simulink model "skarab_fgbe"  (R2016b)
settings: Solver=VariableStepDiscrete  StartTime=0.0  StopTime=50000  RelTol=1e-3
libraries: xbsIndex_r4 x558, casper_library_delays x131, xps_library x5, casper_library_misc x4
(part 3 of 7)

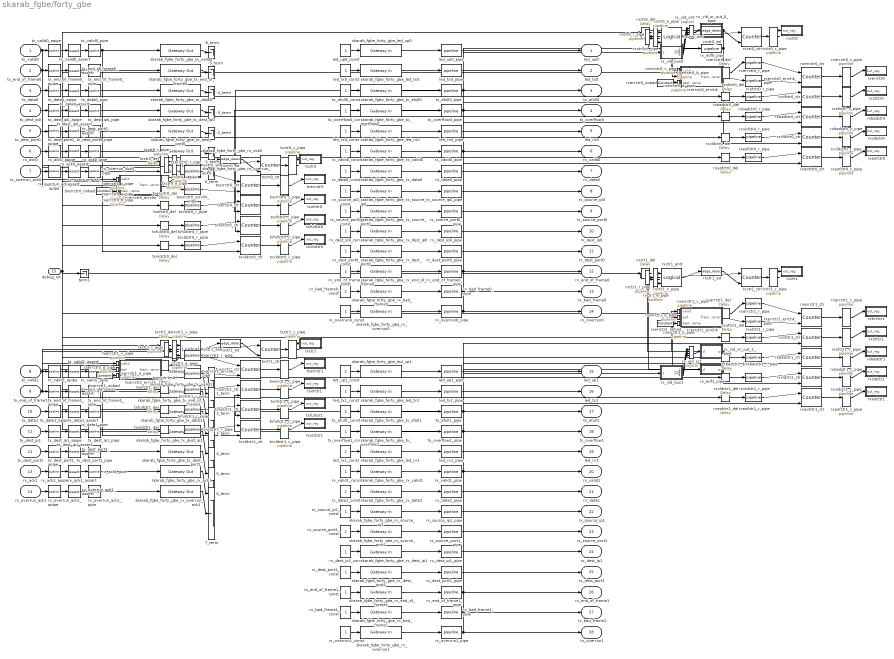
== system skarab_fgbe/forty_gbe ==
  tx_valid0 : Inport
  tx_end_of_frame0 : Inport  Port=2
  tx_data0 : Inport  Port=3
  tx_dest_ip0 : Inport  Port=4
  tx_dest_port0 : Inport  Port=5
  rx_ack0 : Inport  Port=6
  rx_overrun_ack0 : Inport  Port=7
  tx_valid1 : Inport  Port=8
  tx_end_of_frame1 : Inport  Port=9
  tx_data1 : Inport  Port=10
  tx_dest_ip1 : Inport  Port=11
  tx_dest_port1 : Inport  Port=12
  rx_ack1 : Inport  Port=13
  rx_overrun_ack1 : Inport  Port=14
  debug_rst : Inport  Port=15
  -1_term : Terminator
  -2_term : Terminator
  -3_term : Terminator
  -4_term : Terminator
  -5_term : Terminator
  -6_term : Terminator
  0_term : Terminator
  1_term : Terminator
  2_term : Terminator
  3_term : Terminator
  4_term : Terminator
  5_term : Terminator
  6_term : Terminator
  7_term : Terminator
  led_rx0_const : Constant
  led_rx0_pipe : casper_library_delays/pipeline  latency=3
      settings: AttributesFormatString=Latency = %<latency>
  led_rx1_const : Constant
  led_rx1_pipe : casper_library_delays/pipeline  latency=3
      settings: AttributesFormatString=Latency = %<latency>
  led_tx0_const : Constant
  led_tx0_pipe : casper_library_delays/pipeline  latency=3
      settings: AttributesFormatString=Latency = %<latency>
  led_tx1_const : Constant
  led_tx1_pipe : casper_library_delays/pipeline  latency=3
      settings: AttributesFormatString=Latency = %<latency>
  led_up0_const : Constant
  led_up0_pipe : casper_library_delays/pipeline  latency=3
      settings: AttributesFormatString=Latency = %<latency>
  led_up1_const : Constant
  led_up1_pipe : casper_library_delays/pipeline  latency=3
      settings: AttributesFormatString=Latency = %<latency>
  rx_ack0_apipe : casper_library_delays/pipeline  latency=3
      settings: AttributesFormatString=Latency = %<latency>
  rx_ack0_assert : xbsIndex_r4/Assert  assert_type=on  type_source=Explicitly  gui_display_data_type=Fixed-point  arith_type=Boolean  n_bits=1  bin_pt=0  preci_type=Single  exp_width=8  frac_width=24  assert_rate=on  rate_source=Explicitly  period=1  output_port=on  block_type=assert
  rx_ack0_pipe : casper_library_delays/pipeline  latency=3
      settings: AttributesFormatString=Latency = %<latency>
  rx_ack1_apipe : casper_library_delays/pipeline  latency=3
      settings: AttributesFormatString=Latency = %<latency>
  rx_ack1_assert : xbsIndex_r4/Assert  assert_type=on  type_source=Explicitly  gui_display_data_type=Fixed-point  arith_type=Boolean  n_bits=1  bin_pt=0  preci_type=Single  exp_width=8  frac_width=24  assert_rate=on  rate_source=Explicitly  period=1  output_port=on  block_type=assert
  rx_ack1_pipe : casper_library_delays/pipeline  latency=3
      settings: AttributesFormatString=Latency = %<latency>
  rx_bad_frame0_const : Constant
  rx_bad_frame0_pipe : casper_library_delays/pipeline  latency=3
      settings: AttributesFormatString=Latency = %<latency>
  rx_bad_frame1_const : Constant
  rx_bad_frame1_pipe : casper_library_delays/pipeline  latency=3
      settings: AttributesFormatString=Latency = %<latency>
  rx_data0_const : Constant
  rx_data0_pipe : casper_library_delays/pipeline  latency=3
      settings: AttributesFormatString=Latency = %<latency>
  rx_data1_const : Constant
  rx_data1_pipe : casper_library_delays/pipeline  latency=3
      settings: AttributesFormatString=Latency = %<latency>
  rx_dest_ip0_const : Constant
  rx_dest_ip0_pipe : casper_library_delays/pipeline  latency=3
      settings: AttributesFormatString=Latency = %<latency>
  rx_dest_ip1_const : Constant
  rx_dest_ip1_pipe : casper_library_delays/pipeline  latency=3
      settings: AttributesFormatString=Latency = %<latency>
  rx_dest_port0_const : Constant
  rx_dest_port0_pipe : casper_library_delays/pipeline  latency=3
      settings: AttributesFormatString=Latency = %<latency>
  rx_dest_port1_const : Constant
  rx_dest_port1_pipe : casper_library_delays/pipeline  latency=3
      settings: AttributesFormatString=Latency = %<latency>
  rx_end_of_frame0_const : Constant
  rx_end_of_frame0_pipe : casper_library_delays/pipeline  latency=3
      settings: AttributesFormatString=Latency = %<latency>
  rx_end_of_frame1_const : Constant
  rx_end_of_frame1_pipe : casper_library_delays/pipeline  latency=3
      settings: AttributesFormatString=Latency = %<latency>
  rx_eof0_pipe : casper_library_delays/pipeline  latency=3
      settings: AttributesFormatString=Latency = %<latency>
  rx_eof1_pipe : Subsystem  AncestorBlock=casper_library_delays/pipeline  mask(pipeline){latency=3}
      mask help:
      | An explicitly laid-out delay line to avoid mapping to SRL16s
      | for use in pipelining to help achieve timing closure.
      mask init:
      | pipeline_init(gcb,'latency',latency);
      settings: AttributesFormatString=Latency = %<latency>
      mask Display:
      | port_label('input', 1, 'd');
      | port_label('output', 1, 'q');
      | disp(['Z^-', num2str(latency)]);
  rx_overrun0_const : Constant
  rx_overrun0_pipe : casper_library_delays/pipeline  latency=3
      settings: AttributesFormatString=Latency = %<latency>
  rx_overrun1_const : Constant
  rx_overrun1_pipe : casper_library_delays/pipeline  latency=3
      settings: AttributesFormatString=Latency = %<latency>
  rx_overrun_ack0_apipe : casper_library_delays/pipeline  latency=3
      settings: AttributesFormatString=Latency = %<latency>
  rx_overrun_ack0_assert : xbsIndex_r4/Assert  assert_type=on  type_source=Explicitly  gui_display_data_type=Fixed-point  arith_type=Boolean  n_bits=1  bin_pt=0  preci_type=Single  exp_width=8  frac_width=24  assert_rate=on  rate_source=Explicitly  period=1  output_port=on  block_type=assert
  rx_overrun_ack0_pipe : casper_library_delays/pipeline  latency=3
      settings: AttributesFormatString=Latency = %<latency>
  rx_overrun_ack1_apipe : casper_library_delays/pipeline  latency=3
      settings: AttributesFormatString=Latency = %<latency>
  rx_overrun_ack1_assert : xbsIndex_r4/Assert  assert_type=on  type_source=Explicitly  gui_display_data_type=Fixed-point  arith_type=Boolean  n_bits=1  bin_pt=0  preci_type=Single  exp_width=8  frac_width=24  assert_rate=on  rate_source=Explicitly  period=1  output_port=on  block_type=assert
  rx_overrun_ack1_pipe : casper_library_delays/pipeline  latency=3
      settings: AttributesFormatString=Latency = %<latency>
  rx_source_ip0_const : Constant
  rx_source_ip0_pipe : casper_library_delays/pipeline  latency=3
      settings: AttributesFormatString=Latency = %<latency>
  rx_source_ip1_const : Constant
  rx_source_ip1_pipe : casper_library_delays/pipeline  latency=3
      settings: AttributesFormatString=Latency = %<latency>
  rx_source_port0_const : Constant
  rx_source_port0_pipe : casper_library_delays/pipeline  latency=3
      settings: AttributesFormatString=Latency = %<latency>
  rx_source_port1_const : Constant
  rx_source_port1_pipe : casper_library_delays/pipeline  latency=3
      settings: AttributesFormatString=Latency = %<latency>
  rx_valid0_const : Constant
  rx_valid0_pipe : casper_library_delays/pipeline  latency=3
      settings: AttributesFormatString=Latency = %<latency>
  rx_valid1_const : Constant
  rx_valid1_pipe : casper_library_delays/pipeline  latency=3
      settings: AttributesFormatString=Latency = %<latency>
  rx_vld_bus0 : Subsystem  AncestorBlock=casper_library_flow_control/bus_expand  mask(bus_expand){mode=divisions of equal size, outputNum=4, outputWidth=1, outputBinaryPt=0, outputArithmeticType=2, show_format=off, outputToWorkspace=off, variablePrefix=out, outputToModelAsWell=on}
      mask prompts: outputNum "Number of outputs:"; outputWidth "Output width:"; outputBinaryPt "Output binary point position:"; outputArithmeticType "Output arithmetic type (ufix=0, fix=1, bool=2):"; show_format "Print format string?"; outputToWorkspace "Output to workspace?"; variablePrefix "Variable name prefix:"; outputToModelAsWell "Output to model as well?"
      mask help:
      | Expands a 'bus' made using a bus_create or Xilinx
      | concat block.
      | The input will be divided into the specified number
      | of outputs with the specified arithmetic types.
      | Divisions are made from most significant bit.
      mask init:
      | bus_expand_init(gcb,...
      |     'mode', mode, ...
      |     'outputNum', outputNum, ...
      |     'outputWidth', outputWidth, ...
      |     'outputBinaryPt', outputBinaryPt, ...
      |     'outputArithmeticType', outputArithmeticType, ...
      |     'show_format', show_format, ...
      |     'outputToWorkspace', outputToWorkspace, ...
      |     'variablePrefix', variablePrefix, ...
      |     'outputToModelAsWell', outputToModelAsWell);
      settings: AttributesFormatString=4 outputs
      mask TypeOptions mode: divisions of equal size | divisions of arbitrary size
      mask Callback mode: bus_expand_callback();
      mask Callback outputWidth: bus_expand_callback();
      mask Callback outputToWorkspace: bus_expand_callback();
  rx_vld_bus1 : Subsystem  AncestorBlock=casper_library_flow_control/bus_expand  mask(bus_expand){mode=divisions of equal size, outputNum=4, outputWidth=1, outputBinaryPt=0, outputArithmeticType=2, show_format=off, outputToWorkspace=off, variablePrefix=out, outputToModelAsWell=on}
      mask prompts: outputNum "Number of outputs:"; outputWidth "Output width:"; outputBinaryPt "Output binary point position:"; outputArithmeticType "Output arithmetic type (ufix=0, fix=1, bool=2):"; show_format "Print format string?"; outputToWorkspace "Output to workspace?"; variablePrefix "Variable name prefix:"; outputToModelAsWell "Output to model as well?"
      mask help:
      | Expands a 'bus' made using a bus_create or Xilinx
      | concat block.
      | The input will be divided into the specified number
      | of outputs with the specified arithmetic types.
      | Divisions are made from most significant bit.
      mask init: same as skarab_fgbe/forty_gbe/rx_vld_bus0
      settings: AttributesFormatString=4 outputs
      mask TypeOptions mode: divisions of equal size | divisions of arbitrary size
      mask Callback mode: bus_expand_callback();
      mask Callback outputWidth: bus_expand_callback();
      mask Callback outputToWorkspace: bus_expand_callback();
  rx_vld_or0 : xbsIndex_r4/Logical  logical_function=OR  inputs=4  en=off  latency=1  precision=Full  arith_type=Unsigned  n_bits=16  bin_pt=0  align_bp=on  dbl_ovrd=off  block_type=logical
  rx_vld_or1 : xbsIndex_r4/Logical  logical_function=OR  inputs=4  en=off  latency=1  precision=Full  arith_type=Unsigned  n_bits=16  bin_pt=0  align_bp=on  dbl_ovrd=off  block_type=logical
  rx_vld_or_out_0_pipe : Subsystem  AncestorBlock=casper_library_delays/pipeline  mask(pipeline){latency=2}
      mask help:
      | An explicitly laid-out delay line to avoid mapping to SRL16s
      | for use in pipelining to help achieve timing closure.
      mask init:
      | pipeline_init(gcb,'latency',latency);
      settings: AttributesFormatString=Latency = %<latency>
      mask Display:
      | port_label('input', 1, 'd');
      | port_label('output', 1, 'q');
      | disp(['Z^-', num2str(latency)]);
  rx_vld_or_out_1_pipe : Subsystem  AncestorBlock=casper_library_delays/pipeline  mask(pipeline){latency=2}
      mask help:
      | An explicitly laid-out delay line to avoid mapping to SRL16s
      | for use in pipelining to help achieve timing closure.
      mask init:
      | pipeline_init(gcb,'latency',latency);
      settings: AttributesFormatString=Latency = %<latency>
      mask Display:
      | port_label('input', 1, 'd');
      | port_label('output', 1, 'q');
      | disp(['Z^-', num2str(latency)]);
  rxbadctr0 : Subsystem  Tag=xps:sw_reg  AncestorBlock=xps_library/Memory/software_register  mask(swreg){io_dir=To Processor, io_delay=1, init_val=0, sample_period=1, names=reg, bitwidths=16, bin_pts=0, arith_types=0, sim_port=off, show_format=on}
      mask prompts: io_dir "I/O direction"; io_delay "I/O delay"; init_val "Initial Value"; sample_period "Sample period"; names "Bitfield names [msb...lsb]"; bitwidths "Bitfield widths"; bin_pts "Bitfield binary pts"; arith_types "Bitfield types, ufix=0, fix=1, bool=2"; sim_port "Provide sim input/output?"; show_format "Print format string?"
      mask help: A 32-bit software-accessible register. Can be divided into bitfields of varying widths and types using the fields in the block mask.
      mask init:
      | swreg_init(gcb)
      settings: AttributesFormatString=1output:uf16.0 = 16 bits
      mask TypeOptions io_dir: To Processor | From Processor
      mask Callback io_dir:
      | mask_enables = get_param(gcb, 'MaskEnables');
      | mask_names = get_param(gcb, 'MaskNames');
      | if strcmp(get_param(gcb, 'io_dir'), 'To Processor'),
      |     mask_enables{ismember(mask_names, 'sample_period')} = 'off';
      | else
      |     mask_enables{ismember(mask_names, 'sample_period')} = 'on';
      | end
      | set_param(gcb, 'MaskEnables', mask_enables);
      mask DialogControl ParameterTabVar0 Prompt: Setup
  rxbadctr0_c_pipe : casper_library_delays/pipeline  latency=3
      settings: AttributesFormatString=Latency = %<latency>
  rxbadctr0_ctr : xbsIndex_r4/Counter  cnt_type=Free Running  cnt_to=Inf  operation=Up  start_count=0  cnt_by_val=1  arith_type=Unsigned  n_bits=16  bin_pt=0  load_pin=off  rst=on  en=on  explicit_period=on  period=1  use_behavioral_HDL=on  implementation=Fabric  dbl_ovrd=off  block_type=counter
  rxbadctr0_del : xbsIndex_r4/Delay  rst=off  infoeditControl=Selection of Reset will increase slice count due to use of real FFs and instead of SRLs  en=off  latency=1  reg_retiming=on  dbl_ovrd=off  block_type=delay
      settings: infoedit=Hardware notes: A delay line is a chain, each link of which is an SRL16 or SRL32 followed by a flip-flop.
  rxbadctr0_r_pipe : casper_library_delays/pipeline  latency=3
      settings: AttributesFormatString=Latency = %<latency>
  rxbadctr1 : Subsystem  Tag=xps:sw_reg  AncestorBlock=xps_library/Memory/software_register  mask(swreg){io_dir=To Processor, io_delay=1, init_val=0, sample_period=1, names=reg, bitwidths=16, bin_pts=0, arith_types=0, sim_port=off, show_format=on}
      mask prompts: io_dir "I/O direction"; io_delay "I/O delay"; init_val "Initial Value"; sample_period "Sample period"; names "Bitfield names [msb...lsb]"; bitwidths "Bitfield widths"; bin_pts "Bitfield binary pts"; arith_types "Bitfield types, ufix=0, fix=1, bool=2"; sim_port "Provide sim input/output?"; show_format "Print format string?"
      mask help: A 32-bit software-accessible register. Can be divided into bitfields of varying widths and types using the fields in the block mask.
      mask init:
      | swreg_init(gcb)
      settings: AttributesFormatString=1output:uf16.0 = 16 bits
      mask TypeOptions io_dir: To Processor | From Processor
      mask Callback io_dir:
      | mask_enables = get_param(gcb, 'MaskEnables');
      | mask_names = get_param(gcb, 'MaskNames');
      | if strcmp(get_param(gcb, 'io_dir'), 'To Processor'),
      |     mask_enables{ismember(mask_names, 'sample_period')} = 'off';
      | else
      |     mask_enables{ismember(mask_names, 'sample_period')} = 'on';
      | end
      | set_param(gcb, 'MaskEnables', mask_enables);
      mask DialogControl ParameterTabVar0 Prompt: Setup
  rxbadctr1_c_pipe : casper_library_delays/pipeline  latency=3
      settings: AttributesFormatString=Latency = %<latency>
  rxbadctr1_ctr : xbsIndex_r4/Counter  cnt_type=Free Running  cnt_to=Inf  operation=Up  start_count=0  cnt_by_val=1  arith_type=Unsigned  n_bits=16  bin_pt=0  load_pin=off  rst=on  en=on  explicit_period=on  period=1  use_behavioral_HDL=on  implementation=Fabric  dbl_ovrd=off  block_type=counter
  rxbadctr1_del : xbsIndex_r4/Delay  rst=off  infoeditControl=Selection of Reset will increase slice count due to use of real FFs and instead of SRLs  en=off  latency=1  reg_retiming=on  dbl_ovrd=off  block_type=delay
      settings: infoedit=Hardware notes: A delay line is a chain, each link of which is an SRL16 or SRL32 followed by a flip-flop.
  rxbadctr1_r_pipe : casper_library_delays/pipeline  latency=3
      settings: AttributesFormatString=Latency = %<latency>
  rxctr0 : Subsystem  Tag=xps:sw_reg  AncestorBlock=xps_library/Memory/software_register  mask(swreg){io_dir=To Processor, io_delay=1, init_val=0, sample_period=1, names=reg, bitwidths=16, bin_pts=0, arith_types=0, sim_port=off, show_format=on}
      mask prompts: io_dir "I/O direction"; io_delay "I/O delay"; init_val "Initial Value"; sample_period "Sample period"; names "Bitfield names [msb...lsb]"; bitwidths "Bitfield widths"; bin_pts "Bitfield binary pts"; arith_types "Bitfield types, ufix=0, fix=1, bool=2"; sim_port "Provide sim input/output?"; show_format "Print format string?"
      mask help: A 32-bit software-accessible register. Can be divided into bitfields of varying widths and types using the fields in the block mask.
      mask init:
      | swreg_init(gcb)
      settings: AttributesFormatString=1output:uf16.0 = 16 bits
      mask TypeOptions io_dir: To Processor | From Processor
      mask Callback io_dir:
      | mask_enables = get_param(gcb, 'MaskEnables');
      | mask_names = get_param(gcb, 'MaskNames');
      | if strcmp(get_param(gcb, 'io_dir'), 'To Processor'),
      |     mask_enables{ismember(mask_names, 'sample_period')} = 'off';
      | else
      |     mask_enables{ismember(mask_names, 'sample_period')} = 'on';
      | end
      | set_param(gcb, 'MaskEnables', mask_enables);
      mask DialogControl ParameterTabVar0 Prompt: Setup
  rxctr0_and : xbsIndex_r4/Logical  logical_function=AND  inputs=2  en=off  latency=1  precision=Full  arith_type=Unsigned  n_bits=16  bin_pt=0  align_bp=on  dbl_ovrd=off  block_type=logical
  rxctr0_c_pipe : casper_library_delays/pipeline  latency=3
      settings: AttributesFormatString=Latency = %<latency>
  rxctr0_ctr : xbsIndex_r4/Counter  cnt_type=Free Running  cnt_to=Inf  operation=Up  start_count=0  cnt_by_val=1  arith_type=Unsigned  n_bits=16  bin_pt=0  load_pin=off  rst=on  en=on  explicit_period=on  period=1  use_behavioral_HDL=on  implementation=Fabric  dbl_ovrd=off  block_type=counter
  rxctr0_del : xbsIndex_r4/Delay  rst=off  infoeditControl=Selection of Reset will increase slice count due to use of real FFs and instead of SRLs  en=off  latency=1  reg_retiming=on  dbl_ovrd=off  block_type=delay
      settings: infoedit=Hardware notes: A delay line is a chain, each link of which is an SRL16 or SRL32 followed by a flip-flop.
  rxctr0_e_pipe : casper_library_delays/pipeline  latency=3
      settings: AttributesFormatString=Latency = %<latency>
  rxctr0_ed : casper_library_misc/edge_detect  edge=Rising  polarity=Active High  x_in=[0 0.08 0.08 0.16 0.16 0.24 0.24 0.32 0.32 0.4]  y_in="[-1 -1  1  1  1  1  1  1  1  1]"  x_out=[0.6 0.68 0.68 0.76 0.76 0.84 0.84 0.92 0.92 1]  y_out="[-1 -1  1  1 -1 -1 -1 -1 -1 -1]"
  rxctr0_r_pipe : casper_library_delays/pipeline  latency=3
      settings: AttributesFormatString=Latency = %<latency>
  rxctr0_v_pipe : casper_library_delays/pipeline  latency=3
      settings: AttributesFormatString=Latency = %<latency>
  rxctr1 : Subsystem  Tag=xps:sw_reg  AncestorBlock=xps_library/Memory/software_register  mask(swreg){io_dir=To Processor, io_delay=1, init_val=0, sample_period=1, names=reg, bitwidths=16, bin_pts=0, arith_types=0, sim_port=off, show_format=on}
      mask prompts: io_dir "I/O direction"; io_delay "I/O delay"; init_val "Initial Value"; sample_period "Sample period"; names "Bitfield names [msb...lsb]"; bitwidths "Bitfield widths"; bin_pts "Bitfield binary pts"; arith_types "Bitfield types, ufix=0, fix=1, bool=2"; sim_port "Provide sim input/output?"; show_format "Print format string?"
      mask help: A 32-bit software-accessible register. Can be divided into bitfields of varying widths and types using the fields in the block mask.
      mask init:
      | swreg_init(gcb)
      settings: AttributesFormatString=1output:uf16.0 = 16 bits
      mask TypeOptions io_dir: To Processor | From Processor
      mask Callback io_dir:
      | mask_enables = get_param(gcb, 'MaskEnables');
      | mask_names = get_param(gcb, 'MaskNames');
      | if strcmp(get_param(gcb, 'io_dir'), 'To Processor'),
      |     mask_enables{ismember(mask_names, 'sample_period')} = 'off';
      | else
      |     mask_enables{ismember(mask_names, 'sample_period')} = 'on';
      | end
      | set_param(gcb, 'MaskEnables', mask_enables);
      mask DialogControl ParameterTabVar0 Prompt: Setup
  rxctr1_and : xbsIndex_r4/Logical  logical_function=AND  inputs=2  en=off  latency=1  precision=Full  arith_type=Unsigned  n_bits=16  bin_pt=0  align_bp=on  dbl_ovrd=off  block_type=logical
  rxctr1_c_pipe : casper_library_delays/pipeline  latency=3
      settings: AttributesFormatString=Latency = %<latency>
  rxctr1_ctr : xbsIndex_r4/Counter  cnt_type=Free Running  cnt_to=Inf  operation=Up  start_count=0  cnt_by_val=1  arith_type=Unsigned  n_bits=16  bin_pt=0  load_pin=off  rst=on  en=on  explicit_period=on  period=1  use_behavioral_HDL=on  implementation=Fabric  dbl_ovrd=off  block_type=counter
  rxctr1_del : xbsIndex_r4/Delay  rst=off  infoeditControl=Selection of Reset will increase slice count due to use of real FFs and instead of SRLs  en=off  latency=1  reg_retiming=on  dbl_ovrd=off  block_type=delay
      settings: infoedit=Hardware notes: A delay line is a chain, each link of which is an SRL16 or SRL32 followed by a flip-flop.
  rxctr1_e_pipe : casper_library_delays/pipeline  latency=3
      settings: AttributesFormatString=Latency = %<latency>
  rxctr1_ed : casper_library_misc/edge_detect  edge=Rising  polarity=Active High  x_in=[0 0.08 0.08 0.16 0.16 0.24 0.24 0.32 0.32 0.4]  y_in="[-1 -1  1  1  1  1  1  1  1  1]"  x_out=[0.6 0.68 0.68 0.76 0.76 0.84 0.84 0.92 0.92 1]  y_out="[-1 -1  1  1 -1 -1 -1 -1 -1 -1]"
  rxctr1_r_pipe : casper_library_delays/pipeline  latency=3
      settings: AttributesFormatString=Latency = %<latency>
  rxctr1_v_pipe : casper_library_delays/pipeline  latency=3
      settings: AttributesFormatString=Latency = %<latency>
  rxeofctr0 : Subsystem  Tag=xps:sw_reg  AncestorBlock=xps_library/Memory/software_register  mask(swreg){io_dir=To Processor, io_delay=1, init_val=0, sample_period=1, names=reg, bitwidths=16, bin_pts=0, arith_types=0, sim_port=off, show_format=on}
      mask prompts: io_dir "I/O direction"; io_delay "I/O delay"; init_val "Initial Value"; sample_period "Sample period"; names "Bitfield names [msb...lsb]"; bitwidths "Bitfield widths"; bin_pts "Bitfield binary pts"; arith_types "Bitfield types, ufix=0, fix=1, bool=2"; sim_port "Provide sim input/output?"; show_format "Print format string?"
      mask help: A 32-bit software-accessible register. Can be divided into bitfields of varying widths and types using the fields in the block mask.
      mask init:
      | swreg_init(gcb)
      settings: AttributesFormatString=1output:uf16.0 = 16 bits
      mask TypeOptions io_dir: To Processor | From Processor
      mask Callback io_dir:
      | mask_enables = get_param(gcb, 'MaskEnables');
      | mask_names = get_param(gcb, 'MaskNames');
      | if strcmp(get_param(gcb, 'io_dir'), 'To Processor'),
      |     mask_enables{ismember(mask_names, 'sample_period')} = 'off';
      | else
      |     mask_enables{ismember(mask_names, 'sample_period')} = 'on';
      | end
      | set_param(gcb, 'MaskEnables', mask_enables);
      mask DialogControl ParameterTabVar0 Prompt: Setup
  rxeofctr0_c_pipe : casper_library_delays/pipeline  latency=3
      settings: AttributesFormatString=Latency = %<latency>
  rxeofctr0_ctr : xbsIndex_r4/Counter  cnt_type=Free Running  cnt_to=Inf  operation=Up  start_count=0  cnt_by_val=1  arith_type=Unsigned  n_bits=16  bin_pt=0  load_pin=off  rst=on  en=on  explicit_period=on  period=1  use_behavioral_HDL=on  implementation=Fabric  dbl_ovrd=off  block_type=counter
  rxeofctr0_del : xbsIndex_r4/Delay  rst=off  infoeditControl=Selection of Reset will increase slice count due to use of real FFs and instead of SRLs  en=off  latency=1  reg_retiming=on  dbl_ovrd=off  block_type=delay
      settings: infoedit=Hardware notes: A delay line is a chain, each link of which is an SRL16 or SRL32 followed by a flip-flop.
  rxeofctr0_r_pipe : casper_library_delays/pipeline  latency=3
      settings: AttributesFormatString=Latency = %<latency>
  rxeofctr1 : Subsystem  Tag=xps:sw_reg  AncestorBlock=xps_library/Memory/software_register  mask(swreg){io_dir=To Processor, io_delay=1, init_val=0, sample_period=1, names=reg, bitwidths=16, bin_pts=0, arith_types=0, sim_port=off, show_format=on}
      mask prompts: io_dir "I/O direction"; io_delay "I/O delay"; init_val "Initial Value"; sample_period "Sample period"; names "Bitfield names [msb...lsb]"; bitwidths "Bitfield widths"; bin_pts "Bitfield binary pts"; arith_types "Bitfield types, ufix=0, fix=1, bool=2"; sim_port "Provide sim input/output?"; show_format "Print format string?"
      mask help: A 32-bit software-accessible register. Can be divided into bitfields of varying widths and types using the fields in the block mask.
      mask init:
      | swreg_init(gcb)
      settings: AttributesFormatString=1output:uf16.0 = 16 bits
      mask TypeOptions io_dir: To Processor | From Processor
      mask Callback io_dir:
      | mask_enables = get_param(gcb, 'MaskEnables');
      | mask_names = get_param(gcb, 'MaskNames');
      | if strcmp(get_param(gcb, 'io_dir'), 'To Processor'),
      |     mask_enables{ismember(mask_names, 'sample_period')} = 'off';
      | else
      |     mask_enables{ismember(mask_names, 'sample_period')} = 'on';
      | end
      | set_param(gcb, 'MaskEnables', mask_enables);
      mask DialogControl ParameterTabVar0 Prompt: Setup
  rxeofctr1_c_pipe : casper_library_delays/pipeline  latency=3
      settings: AttributesFormatString=Latency = %<latency>
  rxeofctr1_ctr : xbsIndex_r4/Counter  cnt_type=Free Running  cnt_to=Inf  operation=Up  start_count=0  cnt_by_val=1  arith_type=Unsigned  n_bits=16  bin_pt=0  load_pin=off  rst=on  en=on  explicit_period=on  period=1  use_behavioral_HDL=on  implementation=Fabric  dbl_ovrd=off  block_type=counter
  rxeofctr1_del : xbsIndex_r4/Delay  rst=off  infoeditControl=Selection of Reset will increase slice count due to use of real FFs and instead of SRLs  en=off  latency=1  reg_retiming=on  dbl_ovrd=off  block_type=delay
      settings: infoedit=Hardware notes: A delay line is a chain, each link of which is an SRL16 or SRL32 followed by a flip-flop.
  rxeofctr1_r_pipe : casper_library_delays/pipeline  latency=3
      settings: AttributesFormatString=Latency = %<latency>
  rxerrctr0 : Subsystem  Tag=xps:sw_reg  AncestorBlock=xps_library/Memory/software_register  mask(swreg){io_dir=To Processor, io_delay=1, init_val=0, sample_period=1, names=reg, bitwidths=16, bin_pts=0, arith_types=0, sim_port=off, show_format=on}
      mask prompts: io_dir "I/O direction"; io_delay "I/O delay"; init_val "Initial Value"; sample_period "Sample period"; names "Bitfield names [msb...lsb]"; bitwidths "Bitfield widths"; bin_pts "Bitfield binary pts"; arith_types "Bitfield types, ufix=0, fix=1, bool=2"; sim_port "Provide sim input/output?"; show_format "Print format string?"
      mask help: A 32-bit software-accessible register. Can be divided into bitfields of varying widths and types using the fields in the block mask.
      mask init:
      | swreg_init(gcb)
      settings: AttributesFormatString=1output:uf16.0 = 16 bits
      mask TypeOptions io_dir: To Processor | From Processor
      mask Callback io_dir:
      | mask_enables = get_param(gcb, 'MaskEnables');
      | mask_names = get_param(gcb, 'MaskNames');
      | if strcmp(get_param(gcb, 'io_dir'), 'To Processor'),
      |     mask_enables{ismember(mask_names, 'sample_period')} = 'off';
      | else
      |     mask_enables{ismember(mask_names, 'sample_period')} = 'on';
      | end
      | set_param(gcb, 'MaskEnables', mask_enables);
      mask DialogControl ParameterTabVar0 Prompt: Setup
  rxerrctr0_b_pipe : casper_library_delays/pipeline  latency=3
      settings: AttributesFormatString=Latency = %<latency>
  rxerrctr0_c_pipe : casper_library_delays/pipeline  latency=3
      settings: AttributesFormatString=Latency = %<latency>
  rxerrctr0_ctr : xbsIndex_r4/Counter  cnt_type=Free Running  cnt_to=Inf  operation=Up  start_count=0  cnt_by_val=1  arith_type=Unsigned  n_bits=16  bin_pt=0  load_pin=off  rst=on  en=on  explicit_period=on  period=1  use_behavioral_HDL=on  implementation=Fabric  dbl_ovrd=off  block_type=counter
  rxerrctr0_del : xbsIndex_r4/Delay  rst=off  infoeditControl=Selection of Reset will increase slice count due to use of real FFs and instead of SRLs  en=off  latency=1  reg_retiming=on  dbl_ovrd=off  block_type=delay
      settings: infoedit=Hardware notes: A delay line is a chain, each link of which is an SRL16 or SRL32 followed by a flip-flop.
  rxerrctr0_e_pipe : casper_library_delays/pipeline  latency=3
      settings: AttributesFormatString=Latency = %<latency>
  rxerrctr0_errchk : Subsystem  Tag=casper:frame_len_checker  AncestorBlock=casper_library_communications/frame_len_checker  mask{frame_len=100}
      mask prompts: frame_len "Frame length (64-bit words):"
      mask help: Monitors valid, EOF and bad_frame signals in/from a 10Gbe core and outputs an error signal. Can be used to drive an error counter or latched as a flag.
  rxerrctr0_errchk_pipe : casper_library_delays/pipeline  latency=3
      settings: AttributesFormatString=Latency = %<latency>
  rxerrctr0_nobad : xbsIndex_r4/Constant  const=0  gui_display_data_type=Fixed-point  arith_type=Boolean  n_bits=16  bin_pt=14  preci_type=Single  exp_width=8  frac_width=24  explicit_period=on  period=1  equ=P=C  opselect=C  inp2=PCIN>>17  opr=+  inp1=P  carry=CIN  dbl_ovrd=off  block_type=constant
  rxerrctr0_r_pipe : casper_library_delays/pipeline  latency=3
      settings: AttributesFormatString=Latency = %<latency>
  rxerrctr0_v_pipe : casper_library_delays/pipeline  latency=3
      settings: AttributesFormatString=Latency = %<latency>
  rxerrctr1 : Subsystem  Tag=xps:sw_reg  AncestorBlock=xps_library/Memory/software_register  mask(swreg){io_dir=To Processor, io_delay=1, init_val=0, sample_period=1, names=reg, bitwidths=16, bin_pts=0, arith_types=0, sim_port=off, show_format=on}
      mask prompts: io_dir "I/O direction"; io_delay "I/O delay"; init_val "Initial Value"; sample_period "Sample period"; names "Bitfield names [msb...lsb]"; bitwidths "Bitfield widths"; bin_pts "Bitfield binary pts"; arith_types "Bitfield types, ufix=0, fix=1, bool=2"; sim_port "Provide sim input/output?"; show_format "Print format string?"
      mask help: A 32-bit software-accessible register. Can be divided into bitfields of varying widths and types using the fields in the block mask.
      mask init:
      | swreg_init(gcb)
      settings: AttributesFormatString=1output:uf16.0 = 16 bits
      mask TypeOptions io_dir: To Processor | From Processor
      mask Callback io_dir:
      | mask_enables = get_param(gcb, 'MaskEnables');
      | mask_names = get_param(gcb, 'MaskNames');
      | if strcmp(get_param(gcb, 'io_dir'), 'To Processor'),
      |     mask_enables{ismember(mask_names, 'sample_period')} = 'off';
      | else
      |     mask_enables{ismember(mask_names, 'sample_period')} = 'on';
      | end
      | set_param(gcb, 'MaskEnables', mask_enables);
      mask DialogControl ParameterTabVar0 Prompt: Setup
  rxerrctr1_b_pipe : casper_library_delays/pipeline  latency=3
      settings: AttributesFormatString=Latency = %<latency>
  rxerrctr1_c_pipe : casper_library_delays/pipeline  latency=3
      settings: AttributesFormatString=Latency = %<latency>
  rxerrctr1_ctr : xbsIndex_r4/Counter  cnt_type=Free Running  cnt_to=Inf  operation=Up  start_count=0  cnt_by_val=1  arith_type=Unsigned  n_bits=16  bin_pt=0  load_pin=off  rst=on  en=on  explicit_period=on  period=1  use_behavioral_HDL=on  implementation=Fabric  dbl_ovrd=off  block_type=counter
  rxerrctr1_del : xbsIndex_r4/Delay  rst=off  infoeditControl=Selection of Reset will increase slice count due to use of real FFs and instead of SRLs  en=off  latency=1  reg_retiming=on  dbl_ovrd=off  block_type=delay
      settings: infoedit=Hardware notes: A delay line is a chain, each link of which is an SRL16 or SRL32 followed by a flip-flop.
  rxerrctr1_e_pipe : casper_library_delays/pipeline  latency=3
      settings: AttributesFormatString=Latency = %<latency>
  rxerrctr1_errchk : Subsystem  Tag=casper:frame_len_checker  AncestorBlock=casper_library_communications/frame_len_checker  mask{frame_len=100}
      mask prompts: frame_len "Frame length (64-bit words):"
      mask help: Monitors valid, EOF and bad_frame signals in/from a 10Gbe core and outputs an error signal. Can be used to drive an error counter or latched as a flag.
  rxerrctr1_errchk_pipe : casper_library_delays/pipeline  latency=3
      settings: AttributesFormatString=Latency = %<latency>
  rxerrctr1_nobad : xbsIndex_r4/Constant  const=0  gui_display_data_type=Fixed-point  arith_type=Boolean  n_bits=16  bin_pt=14  preci_type=Single  exp_width=8  frac_width=24  explicit_period=on  period=1  equ=P=C  opselect=C  inp2=PCIN>>17  opr=+  inp1=P  carry=CIN  dbl_ovrd=off  block_type=constant
  rxerrctr1_r_pipe : casper_library_delays/pipeline  latency=3
      settings: AttributesFormatString=Latency = %<latency>
  rxerrctr1_v_pipe : casper_library_delays/pipeline  latency=3
      settings: AttributesFormatString=Latency = %<latency>
  rxofctr0 : Subsystem  Tag=xps:sw_reg  AncestorBlock=xps_library/Memory/software_register  mask(swreg){io_dir=To Processor, io_delay=1, init_val=0, sample_period=1, names=reg, bitwidths=16, bin_pts=0, arith_types=0, sim_port=off, show_format=on}
      mask prompts: io_dir "I/O direction"; io_delay "I/O delay"; init_val "Initial Value"; sample_period "Sample period"; names "Bitfield names [msb...lsb]"; bitwidths "Bitfield widths"; bin_pts "Bitfield binary pts"; arith_types "Bitfield types, ufix=0, fix=1, bool=2"; sim_port "Provide sim input/output?"; show_format "Print format string?"
      mask help: A 32-bit software-accessible register. Can be divided into bitfields of varying widths and types using the fields in the block mask.
      mask init:
      | swreg_init(gcb)
      settings: AttributesFormatString=1output:uf16.0 = 16 bits
      mask TypeOptions io_dir: To Processor | From Processor
      mask Callback io_dir:
      | mask_enables = get_param(gcb, 'MaskEnables');
      | mask_names = get_param(gcb, 'MaskNames');
      | if strcmp(get_param(gcb, 'io_dir'), 'To Processor'),
      |     mask_enables{ismember(mask_names, 'sample_period')} = 'off';
      | else
      |     mask_enables{ismember(mask_names, 'sample_period')} = 'on';
      | end
      | set_param(gcb, 'MaskEnables', mask_enables);
      mask DialogControl ParameterTabVar0 Prompt: Setup
  rxofctr0_c_pipe : casper_library_delays/pipeline  latency=3
      settings: AttributesFormatString=Latency = %<latency>
  rxofctr0_ctr : xbsIndex_r4/Counter  cnt_type=Free Running  cnt_to=Inf  operation=Up  start_count=0  cnt_by_val=1  arith_type=Unsigned  n_bits=16  bin_pt=0  load_pin=off  rst=on  en=on  explicit_period=on  period=1  use_behavioral_HDL=on  implementation=Fabric  dbl_ovrd=off  block_type=counter
  rxofctr0_del : xbsIndex_r4/Delay  rst=off  infoeditControl=Selection of Reset will increase slice count due to use of real FFs and instead of SRLs  en=off  latency=1  reg_retiming=on  dbl_ovrd=off  block_type=delay
      settings: infoedit=Hardware notes: A delay line is a chain, each link of which is an SRL16 or SRL32 followed by a flip-flop.
  rxofctr0_r_pipe : casper_library_delays/pipeline  latency=3
      settings: AttributesFormatString=Latency = %<latency>
  rxofctr1 : Subsystem  Tag=xps:sw_reg  AncestorBlock=xps_library/Memory/software_register  mask(swreg){io_dir=To Processor, io_delay=1, init_val=0, sample_period=1, names=reg, bitwidths=16, bin_pts=0, arith_types=0, sim_port=off, show_format=on}
      mask prompts: io_dir "I/O direction"; io_delay "I/O delay"; init_val "Initial Value"; sample_period "Sample period"; names "Bitfield names [msb...lsb]"; bitwidths "Bitfield widths"; bin_pts "Bitfield binary pts"; arith_types "Bitfield types, ufix=0, fix=1, bool=2"; sim_port "Provide sim input/output?"; show_format "Print format string?"
      mask help: A 32-bit software-accessible register. Can be divided into bitfields of varying widths and types using the fields in the block mask.
      mask init:
      | swreg_init(gcb)
      settings: AttributesFormatString=1output:uf16.0 = 16 bits
      mask TypeOptions io_dir: To Processor | From Processor
      mask Callback io_dir:
      | mask_enables = get_param(gcb, 'MaskEnables');
      | mask_names = get_param(gcb, 'MaskNames');
      | if strcmp(get_param(gcb, 'io_dir'), 'To Processor'),
      |     mask_enables{ismember(mask_names, 'sample_period')} = 'off';
      | else
      |     mask_enables{ismember(mask_names, 'sample_period')} = 'on';
      | end
      | set_param(gcb, 'MaskEnables', mask_enables);
      mask DialogControl ParameterTabVar0 Prompt: Setup
  rxofctr1_c_pipe : casper_library_delays/pipeline  latency=3
      settings: AttributesFormatString=Latency = %<latency>
  rxofctr1_ctr : xbsIndex_r4/Counter  cnt_type=Free Running  cnt_to=Inf  operation=Up  start_count=0  cnt_by_val=1  arith_type=Unsigned  n_bits=16  bin_pt=0  load_pin=off  rst=on  en=on  explicit_period=on  period=1  use_behavioral_HDL=on  implementation=Fabric  dbl_ovrd=off  block_type=counter
  rxofctr1_del : xbsIndex_r4/Delay  rst=off  infoeditControl=Selection of Reset will increase slice count due to use of real FFs and instead of SRLs  en=off  latency=1  reg_retiming=on  dbl_ovrd=off  block_type=delay
      settings: infoedit=Hardware notes: A delay line is a chain, each link of which is an SRL16 or SRL32 followed by a flip-flop.
  rxofctr1_r_pipe : casper_library_delays/pipeline  latency=3
      settings: AttributesFormatString=Latency = %<latency>
  rxvldctr0 : Subsystem  Tag=xps:sw_reg  AncestorBlock=xps_library/Memory/software_register  mask(swreg){io_dir=To Processor, io_delay=1, init_val=0, sample_period=1, names=reg, bitwidths=16, bin_pts=0, arith_types=0, sim_port=off, show_format=on}
      mask prompts: io_dir "I/O direction"; io_delay "I/O delay"; init_val "Initial Value"; sample_period "Sample period"; names "Bitfield names [msb...lsb]"; bitwidths "Bitfield widths"; bin_pts "Bitfield binary pts"; arith_types "Bitfield types, ufix=0, fix=1, bool=2"; sim_port "Provide sim input/output?"; show_format "Print format string?"
      mask help: A 32-bit software-accessible register. Can be divided into bitfields of varying widths and types using the fields in the block mask.
      mask init:
      | swreg_init(gcb)
      settings: AttributesFormatString=1output:uf16.0 = 16 bits
      mask TypeOptions io_dir: To Processor | From Processor
      mask Callback io_dir:
      | mask_enables = get_param(gcb, 'MaskEnables');
      | mask_names = get_param(gcb, 'MaskNames');
      | if strcmp(get_param(gcb, 'io_dir'), 'To Processor'),
      |     mask_enables{ismember(mask_names, 'sample_period')} = 'off';
      | else
      |     mask_enables{ismember(mask_names, 'sample_period')} = 'on';
      | end
      | set_param(gcb, 'MaskEnables', mask_enables);
      mask DialogControl ParameterTabVar0 Prompt: Setup
  rxvldctr0_c_pipe : casper_library_delays/pipeline  latency=3
      settings: AttributesFormatString=Latency = %<latency>
  rxvldctr0_ctr : xbsIndex_r4/Counter  cnt_type=Free Running  cnt_to=Inf  operation=Up  start_count=0  cnt_by_val=1  arith_type=Unsigned  n_bits=16  bin_pt=0  load_pin=off  rst=on  en=on  explicit_period=on  period=1  use_behavioral_HDL=on  implementation=Fabric  dbl_ovrd=off  block_type=counter
  rxvldctr0_del : xbsIndex_r4/Delay  rst=off  infoeditControl=Selection of Reset will increase slice count due to use of real FFs and instead of SRLs  en=off  latency=1  reg_retiming=on  dbl_ovrd=off  block_type=delay
      settings: infoedit=Hardware notes: A delay line is a chain, each link of which is an SRL16 or SRL32 followed by a flip-flop.
  rxvldctr0_r_pipe : casper_library_delays/pipeline  latency=3
      settings: AttributesFormatString=Latency = %<latency>
  rxvldctr1 : Subsystem  Tag=xps:sw_reg  AncestorBlock=xps_library/Memory/software_register  mask(swreg){io_dir=To Processor, io_delay=1, init_val=0, sample_period=1, names=reg, bitwidths=16, bin_pts=0, arith_types=0, sim_port=off, show_format=on}
      mask prompts: io_dir "I/O direction"; io_delay "I/O delay"; init_val "Initial Value"; sample_period "Sample period"; names "Bitfield names [msb...lsb]"; bitwidths "Bitfield widths"; bin_pts "Bitfield binary pts"; arith_types "Bitfield types, ufix=0, fix=1, bool=2"; sim_port "Provide sim input/output?"; show_format "Print format string?"
      mask help: A 32-bit software-accessible register. Can be divided into bitfields of varying widths and types using the fields in the block mask.
      mask init:
      | swreg_init(gcb)
      settings: AttributesFormatString=1output:uf16.0 = 16 bits
      mask TypeOptions io_dir: To Processor | From Processor
      mask Callback io_dir:
      | mask_enables = get_param(gcb, 'MaskEnables');
      | mask_names = get_param(gcb, 'MaskNames');
      | if strcmp(get_param(gcb, 'io_dir'), 'To Processor'),
      |     mask_enables{ismember(mask_names, 'sample_period')} = 'off';
      | else
      |     mask_enables{ismember(mask_names, 'sample_period')} = 'on';
      | end
      | set_param(gcb, 'MaskEnables', mask_enables);
      mask DialogControl ParameterTabVar0 Prompt: Setup
  rxvldctr1_c_pipe : casper_library_delays/pipeline  latency=3
      settings: AttributesFormatString=Latency = %<latency>
  rxvldctr1_ctr : xbsIndex_r4/Counter  cnt_type=Free Running  cnt_to=Inf  operation=Up  start_count=0  cnt_by_val=1  arith_type=Unsigned  n_bits=16  bin_pt=0  load_pin=off  rst=on  en=on  explicit_period=on  period=1  use_behavioral_HDL=on  implementation=Fabric  dbl_ovrd=off  block_type=counter
  rxvldctr1_del : xbsIndex_r4/Delay  rst=off  infoeditControl=Selection of Reset will increase slice count due to use of real FFs and instead of SRLs  en=off  latency=1  reg_retiming=on  dbl_ovrd=off  block_type=delay
      settings: infoedit=Hardware notes: A delay line is a chain, each link of which is an SRL16 or SRL32 followed by a flip-flop.
  rxvldctr1_r_pipe : casper_library_delays/pipeline  latency=3
      settings: AttributesFormatString=Latency = %<latency>
  skarab_fgbe_forty_gbe_led_rx0 : xbsIndex_r4/Gateway In  gui_display_data_type=Fixed-point  arith_type=Boolean  n_bits=1  bin_pt=0  preci_type=Single  exp_width=8  frac_width=24  rows=1  columns=1  quantization=Truncate  overflow=Wrap  period=1  UseAsADC=off  ADCChannel='1'  interface=None  automatic_assignment=on  address_offset=hex2dec('00')  intf_name=''  intf_description=''  default_value=0  timing_constraint=None  locs_specified=off  LOCs={}  io_standard={}  inherit_from_input=off  hdl_port=on  dbl_ovrd=off  block_type=gatewayin
  skarab_fgbe_forty_gbe_led_rx1 : xbsIndex_r4/Gateway In  gui_display_data_type=Fixed-point  arith_type=Boolean  n_bits=1  bin_pt=0  preci_type=Single  exp_width=8  frac_width=24  rows=1  columns=1  quantization=Truncate  overflow=Wrap  period=1  UseAsADC=off  ADCChannel='1'  interface=None  automatic_assignment=on  address_offset=hex2dec('00')  intf_name=''  intf_description=''  default_value=0  timing_constraint=None  locs_specified=off  LOCs={}  io_standard={}  inherit_from_input=off  hdl_port=on  dbl_ovrd=off  block_type=gatewayin
  skarab_fgbe_forty_gbe_led_tx0 : xbsIndex_r4/Gateway In  gui_display_data_type=Fixed-point  arith_type=Boolean  n_bits=1  bin_pt=0  preci_type=Single  exp_width=8  frac_width=24  rows=1  columns=1  quantization=Truncate  overflow=Wrap  period=1  UseAsADC=off  ADCChannel='1'  interface=None  automatic_assignment=on  address_offset=hex2dec('00')  intf_name=''  intf_description=''  default_value=0  timing_constraint=None  locs_specified=off  LOCs={}  io_standard={}  inherit_from_input=off  hdl_port=on  dbl_ovrd=off  block_type=gatewayin
  skarab_fgbe_forty_gbe_led_tx1 : xbsIndex_r4/Gateway In  gui_display_data_type=Fixed-point  arith_type=Boolean  n_bits=1  bin_pt=0  preci_type=Single  exp_width=8  frac_width=24  rows=1  columns=1  quantization=Truncate  overflow=Wrap  period=1  UseAsADC=off  ADCChannel='1'  interface=None  automatic_assignment=on  address_offset=hex2dec('00')  intf_name=''  intf_description=''  default_value=0  timing_constraint=None  locs_specified=off  LOCs={}  io_standard={}  inherit_from_input=off  hdl_port=on  dbl_ovrd=off  block_type=gatewayin
  skarab_fgbe_forty_gbe_led_up0 : xbsIndex_r4/Gateway In  gui_display_data_type=Fixed-point  arith_type=Boolean  n_bits=1  bin_pt=0  preci_type=Single  exp_width=8  frac_width=24  rows=1  columns=1  quantization=Truncate  overflow=Wrap  period=1  UseAsADC=off  ADCChannel='1'  interface=None  automatic_assignment=on  address_offset=hex2dec('00')  intf_name=''  intf_description=''  default_value=0  timing_constraint=None  locs_specified=off  LOCs={}  io_standard={}  inherit_from_input=off  hdl_port=on  dbl_ovrd=off  block_type=gatewayin
  skarab_fgbe_forty_gbe_led_up1 : xbsIndex_r4/Gateway In  gui_display_data_type=Fixed-point  arith_type=Boolean  n_bits=1  bin_pt=0  preci_type=Single  exp_width=8  frac_width=24  rows=1  columns=1  quantization=Truncate  overflow=Wrap  period=1  UseAsADC=off  ADCChannel='1'  interface=None  automatic_assignment=on  address_offset=hex2dec('00')  intf_name=''  intf_description=''  default_value=0  timing_constraint=None  locs_specified=off  LOCs={}  io_standard={}  inherit_from_input=off  hdl_port=on  dbl_ovrd=off  block_type=gatewayin
  skarab_fgbe_forty_gbe_rx_ack0 : xbsIndex_r4/Gateway Out  inherit_from_input=off  hdl_port=on  rows=1  columns=1  UseAsDAC=off  DACChannel='1'  interface=None  automatic_assignment=on  address_offset=hex2dec('00')  intf_name=''  intf_description=''  timing_constraint=None  locs_specified=off  LOCs={}  io_standard={}  block_type=gatewayout
  skarab_fgbe_forty_gbe_rx_ack1 : xbsIndex_r4/Gateway Out  inherit_from_input=off  hdl_port=on  rows=1  columns=1  UseAsDAC=off  DACChannel='1'  interface=None  automatic_assignment=on  address_offset=hex2dec('00')  intf_name=''  intf_description=''  timing_constraint=None  locs_specified=off  LOCs={}  io_standard={}  block_type=gatewayout
  skarab_fgbe_forty_gbe_rx_bad_frame0 : xbsIndex_r4/Gateway In  gui_display_data_type=Fixed-point  arith_type=Boolean  n_bits=1  bin_pt=0  preci_type=Single  exp_width=8  frac_width=24  rows=1  columns=1  quantization=Truncate  overflow=Wrap  period=1  UseAsADC=off  ADCChannel='1'  interface=None  automatic_assignment=on  address_offset=hex2dec('00')  intf_name=''  intf_description=''  default_value=0  timing_constraint=None  locs_specified=off  LOCs={}  io_standard={}  inherit_from_input=off  hdl_port=on  dbl_ovrd=off  block_type=gatewayin
  skarab_fgbe_forty_gbe_rx_bad_frame1 : xbsIndex_r4/Gateway In  gui_display_data_type=Fixed-point  arith_type=Boolean  n_bits=1  bin_pt=0  preci_type=Single  exp_width=8  frac_width=24  rows=1  columns=1  quantization=Truncate  overflow=Wrap  period=1  UseAsADC=off  ADCChannel='1'  interface=None  automatic_assignment=on  address_offset=hex2dec('00')  intf_name=''  intf_description=''  default_value=0  timing_constraint=None  locs_specified=off  LOCs={}  io_standard={}  inherit_from_input=off  hdl_port=on  dbl_ovrd=off  block_type=gatewayin
  skarab_fgbe_forty_gbe_rx_data0 : xbsIndex_r4/Gateway In  gui_display_data_type=Fixed-point  arith_type=Unsigned  n_bits=256  bin_pt=0  preci_type=Single  exp_width=8  frac_width=24  rows=1  columns=1  quantization=Truncate  overflow=Wrap  period=1  UseAsADC=off  ADCChannel='1'  interface=None  automatic_assignment=on  address_offset=hex2dec('00')  intf_name=''  intf_description=''  default_value=0  timing_constraint=None  locs_specified=off  LOCs={}  io_standard={}  inherit_from_input=off  hdl_port=on  dbl_ovrd=off  block_type=gatewayin
  skarab_fgbe_forty_gbe_rx_data1 : xbsIndex_r4/Gateway In  gui_display_data_type=Fixed-point  arith_type=Unsigned  n_bits=256  bin_pt=0  preci_type=Single  exp_width=8  frac_width=24  rows=1  columns=1  quantization=Truncate  overflow=Wrap  period=1  UseAsADC=off  ADCChannel='1'  interface=None  automatic_assignment=on  address_offset=hex2dec('00')  intf_name=''  intf_description=''  default_value=0  timing_constraint=None  locs_specified=off  LOCs={}  io_standard={}  inherit_from_input=off  hdl_port=on  dbl_ovrd=off  block_type=gatewayin
  skarab_fgbe_forty_gbe_rx_dest_ip0 : xbsIndex_r4/Gateway In  gui_display_data_type=Fixed-point  arith_type=Unsigned  n_bits=32  bin_pt=0  preci_type=Single  exp_width=8  frac_width=24  rows=1  columns=1  quantization=Truncate  overflow=Wrap  period=1  UseAsADC=off  ADCChannel='1'  interface=None  automatic_assignment=on  address_offset=hex2dec('00')  intf_name=''  intf_description=''  default_value=0  timing_constraint=None  locs_specified=off  LOCs={}  io_standard={}  inherit_from_input=off  hdl_port=on  dbl_ovrd=off  block_type=gatewayin
  skarab_fgbe_forty_gbe_rx_dest_ip1 : xbsIndex_r4/Gateway In  gui_display_data_type=Fixed-point  arith_type=Unsigned  n_bits=32  bin_pt=0  preci_type=Single  exp_width=8  frac_width=24  rows=1  columns=1  quantization=Truncate  overflow=Wrap  period=1  UseAsADC=off  ADCChannel='1'  interface=None  automatic_assignment=on  address_offset=hex2dec('00')  intf_name=''  intf_description=''  default_value=0  timing_constraint=None  locs_specified=off  LOCs={}  io_standard={}  inherit_from_input=off  hdl_port=on  dbl_ovrd=off  block_type=gatewayin
  skarab_fgbe_forty_gbe_rx_dest_port0 : xbsIndex_r4/Gateway In  gui_display_data_type=Fixed-point  arith_type=Unsigned  n_bits=16  bin_pt=0  preci_type=Single  exp_width=8  frac_width=24  rows=1  columns=1  quantization=Truncate  overflow=Wrap  period=1  UseAsADC=off  ADCChannel='1'  interface=None  automatic_assignment=on  address_offset=hex2dec('00')  intf_name=''  intf_description=''  default_value=0  timing_constraint=None  locs_specified=off  LOCs={}  io_standard={}  inherit_from_input=off  hdl_port=on  dbl_ovrd=off  block_type=gatewayin
  skarab_fgbe_forty_gbe_rx_dest_port1 : xbsIndex_r4/Gateway In  gui_display_data_type=Fixed-point  arith_type=Unsigned  n_bits=16  bin_pt=0  preci_type=Single  exp_width=8  frac_width=24  rows=1  columns=1  quantization=Truncate  overflow=Wrap  period=1  UseAsADC=off  ADCChannel='1'  interface=None  automatic_assignment=on  address_offset=hex2dec('00')  intf_name=''  intf_description=''  default_value=0  timing_constraint=None  locs_specified=off  LOCs={}  io_standard={}  inherit_from_input=off  hdl_port=on  dbl_ovrd=off  block_type=gatewayin
  skarab_fgbe_forty_gbe_rx_end_of_frame0 : xbsIndex_r4/Gateway In  gui_display_data_type=Fixed-point  arith_type=Boolean  n_bits=1  bin_pt=0  preci_type=Single  exp_width=8  frac_width=24  rows=1  columns=1  quantization=Truncate  overflow=Wrap  period=1  UseAsADC=off  ADCChannel='1'  interface=None  automatic_assignment=on  address_offset=hex2dec('00')  intf_name=''  intf_description=''  default_value=0  timing_constraint=None  locs_specified=off  LOCs={}  io_standard={}  inherit_from_input=off  hdl_port=on  dbl_ovrd=off  block_type=gatewayin
  skarab_fgbe_forty_gbe_rx_end_of_frame1 : xbsIndex_r4/Gateway In  gui_display_data_type=Fixed-point  arith_type=Boolean  n_bits=1  bin_pt=0  preci_type=Single  exp_width=8  frac_width=24  rows=1  columns=1  quantization=Truncate  overflow=Wrap  period=1  UseAsADC=off  ADCChannel='1'  interface=None  automatic_assignment=on  address_offset=hex2dec('00')  intf_name=''  intf_description=''  default_value=0  timing_constraint=None  locs_specified=off  LOCs={}  io_standard={}  inherit_from_input=off  hdl_port=on  dbl_ovrd=off  block_type=gatewayin
  skarab_fgbe_forty_gbe_rx_overrun0 : xbsIndex_r4/Gateway In  gui_display_data_type=Fixed-point  arith_type=Boolean  n_bits=1  bin_pt=0  preci_type=Single  exp_width=8  frac_width=24  rows=1  columns=1  quantization=Truncate  overflow=Wrap  period=1  UseAsADC=off  ADCChannel='1'  interface=None  automatic_assignment=on  address_offset=hex2dec('00')  intf_name=''  intf_description=''  default_value=0  timing_constraint=None  locs_specified=off  LOCs={}  io_standard={}  inherit_from_input=off  hdl_port=on  dbl_ovrd=off  block_type=gatewayin
  skarab_fgbe_forty_gbe_rx_overrun1 : xbsIndex_r4/Gateway In  gui_display_data_type=Fixed-point  arith_type=Boolean  n_bits=1  bin_pt=0  preci_type=Single  exp_width=8  frac_width=24  rows=1  columns=1  quantization=Truncate  overflow=Wrap  period=1  UseAsADC=off  ADCChannel='1'  interface=None  automatic_assignment=on  address_offset=hex2dec('00')  intf_name=''  intf_description=''  default_value=0  timing_constraint=None  locs_specified=off  LOCs={}  io_standard={}  inherit_from_input=off  hdl_port=on  dbl_ovrd=off  block_type=gatewayin
  skarab_fgbe_forty_gbe_rx_overrun_ack0 : xbsIndex_r4/Gateway Out  inherit_from_input=off  hdl_port=on  rows=1  columns=1  UseAsDAC=off  DACChannel='1'  interface=None  automatic_assignment=on  address_offset=hex2dec('00')  intf_name=''  intf_description=''  timing_constraint=None  locs_specified=off  LOCs={}  io_standard={}  block_type=gatewayout
  skarab_fgbe_forty_gbe_rx_overrun_ack1 : xbsIndex_r4/Gateway Out  inherit_from_input=off  hdl_port=on  rows=1  columns=1  UseAsDAC=off  DACChannel='1'  interface=None  automatic_assignment=on  address_offset=hex2dec('00')  intf_name=''  intf_description=''  timing_constraint=None  locs_specified=off  LOCs={}  io_standard={}  block_type=gatewayout
  skarab_fgbe_forty_gbe_rx_source_ip0 : xbsIndex_r4/Gateway In  gui_display_data_type=Fixed-point  arith_type=Unsigned  n_bits=32  bin_pt=0  preci_type=Single  exp_width=8  frac_width=24  rows=1  columns=1  quantization=Truncate  overflow=Wrap  period=1  UseAsADC=off  ADCChannel='1'  interface=None  automatic_assignment=on  address_offset=hex2dec('00')  intf_name=''  intf_description=''  default_value=0  timing_constraint=None  locs_specified=off  LOCs={}  io_standard={}  inherit_from_input=off  hdl_port=on  dbl_ovrd=off  block_type=gatewayin
  skarab_fgbe_forty_gbe_rx_source_ip1 : xbsIndex_r4/Gateway In  gui_display_data_type=Fixed-point  arith_type=Unsigned  n_bits=32  bin_pt=0  preci_type=Single  exp_width=8  frac_width=24  rows=1  columns=1  quantization=Truncate  overflow=Wrap  period=1  UseAsADC=off  ADCChannel='1'  interface=None  automatic_assignment=on  address_offset=hex2dec('00')  intf_name=''  intf_description=''  default_value=0  timing_constraint=None  locs_specified=off  LOCs={}  io_standard={}  inherit_from_input=off  hdl_port=on  dbl_ovrd=off  block_type=gatewayin
  skarab_fgbe_forty_gbe_rx_source_port0 : xbsIndex_r4/Gateway In  gui_display_data_type=Fixed-point  arith_type=Unsigned  n_bits=16  bin_pt=0  preci_type=Single  exp_width=8  frac_width=24  rows=1  columns=1  quantization=Truncate  overflow=Wrap  period=1  UseAsADC=off  ADCChannel='1'  interface=None  automatic_assignment=on  address_offset=hex2dec('00')  intf_name=''  intf_description=''  default_value=0  timing_constraint=None  locs_specified=off  LOCs={}  io_standard={}  inherit_from_input=off  hdl_port=on  dbl_ovrd=off  block_type=gatewayin
  skarab_fgbe_forty_gbe_rx_source_port1 : xbsIndex_r4/Gateway In  gui_display_data_type=Fixed-point  arith_type=Unsigned  n_bits=16  bin_pt=0  preci_type=Single  exp_width=8  frac_width=24  rows=1  columns=1  quantization=Truncate  overflow=Wrap  period=1  UseAsADC=off  ADCChannel='1'  interface=None  automatic_assignment=on  address_offset=hex2dec('00')  intf_name=''  intf_description=''  default_value=0  timing_constraint=None  locs_specified=off  LOCs={}  io_standard={}  inherit_from_input=off  hdl_port=on  dbl_ovrd=off  block_type=gatewayin
  skarab_fgbe_forty_gbe_rx_valid0 : xbsIndex_r4/Gateway In  gui_display_data_type=Fixed-point  arith_type=Unsigned  n_bits=4  bin_pt=0  preci_type=Single  exp_width=8  frac_width=24  rows=1  columns=1  quantization=Truncate  overflow=Wrap  period=1  UseAsADC=off  ADCChannel='1'  interface=None  automatic_assignment=on  address_offset=hex2dec('00')  intf_name=''  intf_description=''  default_value=0  timing_constraint=None  locs_specified=off  LOCs={}  io_standard={}  inherit_from_input=off  hdl_port=on  dbl_ovrd=off  block_type=gatewayin
  skarab_fgbe_forty_gbe_rx_valid1 : xbsIndex_r4/Gateway In  gui_display_data_type=Fixed-point  arith_type=Unsigned  n_bits=4  bin_pt=0  preci_type=Single  exp_width=8  frac_width=24  rows=1  columns=1  quantization=Truncate  overflow=Wrap  period=1  UseAsADC=off  ADCChannel='1'  interface=None  automatic_assignment=on  address_offset=hex2dec('00')  intf_name=''  intf_description=''  default_value=0  timing_constraint=None  locs_specified=off  LOCs={}  io_standard={}  inherit_from_input=off  hdl_port=on  dbl_ovrd=off  block_type=gatewayin
  skarab_fgbe_forty_gbe_tx_afull0 : xbsIndex_r4/Gateway In  gui_display_data_type=Fixed-point  arith_type=Boolean  n_bits=1  bin_pt=0  preci_type=Single  exp_width=8  frac_width=24  rows=1  columns=1  quantization=Truncate  overflow=Wrap  period=1  UseAsADC=off  ADCChannel='1'  interface=None  automatic_assignment=on  address_offset=hex2dec('00')  intf_name=''  intf_description=''  default_value=0  timing_constraint=None  locs_specified=off  LOCs={}  io_standard={}  inherit_from_input=off  hdl_port=on  dbl_ovrd=off  block_type=gatewayin
  skarab_fgbe_forty_gbe_tx_afull1 : xbsIndex_r4/Gateway In  gui_display_data_type=Fixed-point  arith_type=Boolean  n_bits=1  bin_pt=0  preci_type=Single  exp_width=8  frac_width=24  rows=1  columns=1  quantization=Truncate  overflow=Wrap  period=1  UseAsADC=off  ADCChannel='1'  interface=None  automatic_assignment=on  address_offset=hex2dec('00')  intf_name=''  intf_description=''  default_value=0  timing_constraint=None  locs_specified=off  LOCs={}  io_standard={}  inherit_from_input=off  hdl_port=on  dbl_ovrd=off  block_type=gatewayin
  skarab_fgbe_forty_gbe_tx_data0 : xbsIndex_r4/Gateway Out  inherit_from_input=off  hdl_port=on  rows=1  columns=1  UseAsDAC=off  DACChannel='1'  interface=None  automatic_assignment=on  address_offset=hex2dec('00')  intf_name=''  intf_description=''  timing_constraint=None  locs_specified=off  LOCs={}  io_standard={}  block_type=gatewayout
  skarab_fgbe_forty_gbe_tx_data1 : xbsIndex_r4/Gateway Out  inherit_from_input=off  hdl_port=on  rows=1  columns=1  UseAsDAC=off  DACChannel='1'  interface=None  automatic_assignment=on  address_offset=hex2dec('00')  intf_name=''  intf_description=''  timing_constraint=None  locs_specified=off  LOCs={}  io_standard={}  block_type=gatewayout
  skarab_fgbe_forty_gbe_tx_dest_ip0 : xbsIndex_r4/Gateway Out  inherit_from_input=off  hdl_port=on  rows=1  columns=1  UseAsDAC=off  DACChannel='1'  interface=None  automatic_assignment=on  address_offset=hex2dec('00')  intf_name=''  intf_description=''  timing_constraint=None  locs_specified=off  LOCs={}  io_standard={}  block_type=gatewayout
  skarab_fgbe_forty_gbe_tx_dest_ip1 : xbsIndex_r4/Gateway Out  inherit_from_input=off  hdl_port=on  rows=1  columns=1  UseAsDAC=off  DACChannel='1'  interface=None  automatic_assignment=on  address_offset=hex2dec('00')  intf_name=''  intf_description=''  timing_constraint=None  locs_specified=off  LOCs={}  io_standard={}  block_type=gatewayout
  skarab_fgbe_forty_gbe_tx_dest_port0 : xbsIndex_r4/Gateway Out  inherit_from_input=off  hdl_port=on  rows=1  columns=1  UseAsDAC=off  DACChannel='1'  interface=None  automatic_assignment=on  address_offset=hex2dec('00')  intf_name=''  intf_description=''  timing_constraint=None  locs_specified=off  LOCs={}  io_standard={}  block_type=gatewayout
  skarab_fgbe_forty_gbe_tx_dest_port1 : xbsIndex_r4/Gateway Out  inherit_from_input=off  hdl_port=on  rows=1  columns=1  UseAsDAC=off  DACChannel='1'  interface=None  automatic_assignment=on  address_offset=hex2dec('00')  intf_name=''  intf_description=''  timing_constraint=None  locs_specified=off  LOCs={}  io_standard={}  block_type=gatewayout
  skarab_fgbe_forty_gbe_tx_end_of_frame0 : xbsIndex_r4/Gateway Out  inherit_from_input=off  hdl_port=on  rows=1  columns=1  UseAsDAC=off  DACChannel='1'  interface=None  automatic_assignment=on  address_offset=hex2dec('00')  intf_name=''  intf_description=''  timing_constraint=None  locs_specified=off  LOCs={}  io_standard={}  block_type=gatewayout
  skarab_fgbe_forty_gbe_tx_end_of_frame1 : xbsIndex_r4/Gateway Out  inherit_from_input=off  hdl_port=on  rows=1  columns=1  UseAsDAC=off  DACChannel='1'  interface=None  automatic_assignment=on  address_offset=hex2dec('00')  intf_name=''  intf_description=''  timing_constraint=None  locs_specified=off  LOCs={}  io_standard={}  block_type=gatewayout
  skarab_fgbe_forty_gbe_tx_overflow0 : xbsIndex_r4/Gateway In  gui_display_data_type=Fixed-point  arith_type=Boolean  n_bits=1  bin_pt=0  preci_type=Single  exp_width=8  frac_width=24  rows=1  columns=1  quantization=Truncate  overflow=Wrap  period=1  UseAsADC=off  ADCChannel='1'  interface=None  automatic_assignment=on  address_offset=hex2dec('00')  intf_name=''  intf_description=''  default_value=0  timing_constraint=None  locs_specified=off  LOCs={}  io_standard={}  inherit_from_input=off  hdl_port=on  dbl_ovrd=off  block_type=gatewayin
  skarab_fgbe_forty_gbe_tx_overflow1 : xbsIndex_r4/Gateway In  gui_display_data_type=Fixed-point  arith_type=Boolean  n_bits=1  bin_pt=0  preci_type=Single  exp_width=8  frac_width=24  rows=1  columns=1  quantization=Truncate  overflow=Wrap  period=1  UseAsADC=off  ADCChannel='1'  interface=None  automatic_assignment=on  address_offset=hex2dec('00')  intf_name=''  intf_description=''  default_value=0  timing_constraint=None  locs_specified=off  LOCs={}  io_standard={}  inherit_from_input=off  hdl_port=on  dbl_ovrd=off  block_type=gatewayin
  skarab_fgbe_forty_gbe_tx_valid0 : xbsIndex_r4/Gateway Out  inherit_from_input=off  hdl_port=on  rows=1  columns=1  UseAsDAC=off  DACChannel='1'  interface=None  automatic_assignment=on  address_offset=hex2dec('00')  intf_name=''  intf_description=''  timing_constraint=None  locs_specified=off  LOCs={}  io_standard={}  block_type=gatewayout
  skarab_fgbe_forty_gbe_tx_valid1 : xbsIndex_r4/Gateway Out  inherit_from_input=off  hdl_port=on  rows=1  columns=1  UseAsDAC=off  DACChannel='1'  interface=None  automatic_assignment=on  address_offset=hex2dec('00')  intf_name=''  intf_description=''  timing_constraint=None  locs_specified=off  LOCs={}  io_standard={}  block_type=gatewayout
  term1 : Terminator
  tx_afull0_const : Constant
  tx_afull0_pipe : casper_library_delays/pipeline  latency=3
      settings: AttributesFormatString=Latency = %<latency>
  tx_afull1_const : Constant
  tx_afull1_pipe : casper_library_delays/pipeline  latency=3
      settings: AttributesFormatString=Latency = %<latency>
  tx_data0_apipe : casper_library_delays/pipeline  latency=3
      settings: AttributesFormatString=Latency = %<latency>
  tx_data0_assert : xbsIndex_r4/Assert  assert_type=on  type_source=Explicitly  gui_display_data_type=Fixed-point  arith_type=Unsigned  n_bits=256  bin_pt=0  preci_type=Single  exp_width=8  frac_width=24  assert_rate=on  rate_source=Explicitly  period=1  output_port=on  block_type=assert
  tx_data0_pipe : casper_library_delays/pipeline  latency=3
      settings: AttributesFormatString=Latency = %<latency>
  tx_data1_apipe : casper_library_delays/pipeline  latency=3
      settings: AttributesFormatString=Latency = %<latency>
  tx_data1_assert : xbsIndex_r4/Assert  assert_type=on  type_source=Explicitly  gui_display_data_type=Fixed-point  arith_type=Unsigned  n_bits=256  bin_pt=0  preci_type=Single  exp_width=8  frac_width=24  assert_rate=on  rate_source=Explicitly  period=1  output_port=on  block_type=assert
  tx_data1_pipe : casper_library_delays/pipeline  latency=3
      settings: AttributesFormatString=Latency = %<latency>
  tx_dest_ip0_apipe : casper_library_delays/pipeline  latency=3
      settings: AttributesFormatString=Latency = %<latency>
  tx_dest_ip0_assert : xbsIndex_r4/Assert  assert_type=on  type_source=Explicitly  gui_display_data_type=Fixed-point  arith_type=Unsigned  n_bits=32  bin_pt=0  preci_type=Single  exp_width=8  frac_width=24  assert_rate=on  rate_source=Explicitly  period=1  output_port=on  block_type=assert
  tx_dest_ip0_pipe : casper_library_delays/pipeline  latency=3
      settings: AttributesFormatString=Latency = %<latency>
  tx_dest_ip1_apipe : casper_library_delays/pipeline  latency=3
      settings: AttributesFormatString=Latency = %<latency>
  tx_dest_ip1_assert : xbsIndex_r4/Assert  assert_type=on  type_source=Explicitly  gui_display_data_type=Fixed-point  arith_type=Unsigned  n_bits=32  bin_pt=0  preci_type=Single  exp_width=8  frac_width=24  assert_rate=on  rate_source=Explicitly  period=1  output_port=on  block_type=assert
  tx_dest_ip1_pipe : casper_library_delays/pipeline  latency=3
      settings: AttributesFormatString=Latency = %<latency>
  tx_dest_port0_apipe : casper_library_delays/pipeline  latency=3
      settings: AttributesFormatString=Latency = %<latency>
  tx_dest_port0_assert : xbsIndex_r4/Assert  assert_type=on  type_source=Explicitly  gui_display_data_type=Fixed-point  arith_type=Unsigned  n_bits=16  bin_pt=0  preci_type=Single  exp_width=8  frac_width=24  assert_rate=on  rate_source=Explicitly  period=1  output_port=on  block_type=assert
  tx_dest_port0_pipe : casper_library_delays/pipeline  latency=3
      settings: AttributesFormatString=Latency = %<latency>
  tx_dest_port1_apipe : casper_library_delays/pipeline  latency=3
      settings: AttributesFormatString=Latency = %<latency>
  tx_dest_port1_assert : xbsIndex_r4/Assert  assert_type=on  type_source=Explicitly  gui_display_data_type=Fixed-point  arith_type=Unsigned  n_bits=16  bin_pt=0  preci_type=Single  exp_width=8  frac_width=24  assert_rate=on  rate_source=Explicitly  period=1  output_port=on  block_type=assert
  tx_dest_port1_pipe : casper_library_delays/pipeline  latency=3
      settings: AttributesFormatString=Latency = %<latency>
  tx_end_of_frame0_apipe : casper_library_delays/pipeline  latency=3
      settings: AttributesFormatString=Latency = %<latency>
  tx_end_of_frame0_assert : xbsIndex_r4/Assert  assert_type=on  type_source=Explicitly  gui_display_data_type=Fixed-point  arith_type=Boolean  n_bits=1  bin_pt=0  preci_type=Single  exp_width=8  frac_width=24  assert_rate=on  rate_source=Explicitly  period=1  output_port=on  block_type=assert
  tx_end_of_frame0_pipe : casper_library_delays/pipeline  latency=3
      settings: AttributesFormatString=Latency = %<latency>
  tx_end_of_frame1_apipe : casper_library_delays/pipeline  latency=3
      settings: AttributesFormatString=Latency = %<latency>
  tx_end_of_frame1_assert : xbsIndex_r4/Assert  assert_type=on  type_source=Explicitly  gui_display_data_type=Fixed-point  arith_type=Boolean  n_bits=1  bin_pt=0  preci_type=Single  exp_width=8  frac_width=24  assert_rate=on  rate_source=Explicitly  period=1  output_port=on  block_type=assert
  tx_end_of_frame1_pipe : casper_library_delays/pipeline  latency=3
      settings: AttributesFormatString=Latency = %<latency>
  tx_overflow0_const : Constant
  tx_overflow0_pipe : casper_library_delays/pipeline  latency=3
      settings: AttributesFormatString=Latency = %<latency>
  tx_overflow1_const : Constant
  tx_overflow1_pipe : casper_library_delays/pipeline  latency=3
      settings: AttributesFormatString=Latency = %<latency>
  tx_valid0_apipe : casper_library_delays/pipeline  latency=3
      settings: AttributesFormatString=Latency = %<latency>
  tx_valid0_assert : xbsIndex_r4/Assert  assert_type=on  type_source=Explicitly  gui_display_data_type=Fixed-point  arith_type=Boolean  n_bits=1  bin_pt=0  preci_type=Single  exp_width=8  frac_width=24  assert_rate=on  rate_source=Explicitly  period=1  output_port=on  block_type=assert
  tx_valid0_pipe : casper_library_delays/pipeline  latency=3
      settings: AttributesFormatString=Latency = %<latency>
  tx_valid1_apipe : casper_library_delays/pipeline  latency=3
      settings: AttributesFormatString=Latency = %<latency>
  tx_valid1_assert : xbsIndex_r4/Assert  assert_type=on  type_source=Explicitly  gui_display_data_type=Fixed-point  arith_type=Boolean  n_bits=1  bin_pt=0  preci_type=Single  exp_width=8  frac_width=24  assert_rate=on  rate_source=Explicitly  period=1  output_port=on  block_type=assert
  tx_valid1_pipe : casper_library_delays/pipeline  latency=3
      settings: AttributesFormatString=Latency = %<latency>
  txctr0 : Subsystem  Tag=xps:sw_reg  AncestorBlock=xps_library/Memory/software_register  mask(swreg){io_dir=To Processor, io_delay=1, init_val=0, sample_period=1, names=reg, bitwidths=16, bin_pts=0, arith_types=0, sim_port=off, show_format=on}
      mask prompts: io_dir "I/O direction"; io_delay "I/O delay"; init_val "Initial Value"; sample_period "Sample period"; names "Bitfield names [msb...lsb]"; bitwidths "Bitfield widths"; bin_pts "Bitfield binary pts"; arith_types "Bitfield types, ufix=0, fix=1, bool=2"; sim_port "Provide sim input/output?"; show_format "Print format string?"
      mask help: A 32-bit software-accessible register. Can be divided into bitfields of varying widths and types using the fields in the block mask.
      mask init:
      | swreg_init(gcb)
      settings: AttributesFormatString=1output:uf16.0 = 16 bits
      mask TypeOptions io_dir: To Processor | From Processor
      mask Callback io_dir:
      | mask_enables = get_param(gcb, 'MaskEnables');
      | mask_names = get_param(gcb, 'MaskNames');
      | if strcmp(get_param(gcb, 'io_dir'), 'To Processor'),
      |     mask_enables{ismember(mask_names, 'sample_period')} = 'off';
      | else
      |     mask_enables{ismember(mask_names, 'sample_period')} = 'on';
      | end
      | set_param(gcb, 'MaskEnables', mask_enables);
      mask DialogControl ParameterTabVar0 Prompt: Setup
  txctr0_and : xbsIndex_r4/Logical  logical_function=AND  inputs=2  en=off  latency=1  precision=Full  arith_type=Unsigned  n_bits=16  bin_pt=0  align_bp=on  dbl_ovrd=off  block_type=logical
  txctr0_c_pipe : casper_library_delays/pipeline  latency=3
      settings: AttributesFormatString=Latency = %<latency>
  txctr0_ctr : xbsIndex_r4/Counter  cnt_type=Free Running  cnt_to=Inf  operation=Up  start_count=0  cnt_by_val=1  arith_type=Unsigned  n_bits=16  bin_pt=0  load_pin=off  rst=on  en=on  explicit_period=on  period=1  use_behavioral_HDL=on  implementation=Fabric  dbl_ovrd=off  block_type=counter
  txctr0_del : xbsIndex_r4/Delay  rst=off  infoeditControl=Selection of Reset will increase slice count due to use of real FFs and instead of SRLs  en=off  latency=1  reg_retiming=on  dbl_ovrd=off  block_type=delay
      settings: infoedit=Hardware notes: A delay line is a chain, each link of which is an SRL16 or SRL32 followed by a flip-flop.
  txctr0_e_pipe : casper_library_delays/pipeline  latency=3
      settings: AttributesFormatString=Latency = %<latency>
  txctr0_ed : casper_library_misc/edge_detect  edge=Rising  polarity=Active High  x_in=[0 0.08 0.08 0.16 0.16 0.24 0.24 0.32 0.32 0.4]  y_in="[-1 -1  1  1  1  1  1  1  1  1]"  x_out=[0.6 0.68 0.68 0.76 0.76 0.84 0.84 0.92 0.92 1]  y_out="[-1 -1  1  1 -1 -1 -1 -1 -1 -1]"
  txctr0_r_pipe : casper_library_delays/pipeline  latency=3
      settings: AttributesFormatString=Latency = %<latency>
  txctr0_v_pipe : casper_library_delays/pipeline  latency=3
      settings: AttributesFormatString=Latency = %<latency>
  txctr1 : Subsystem  Tag=xps:sw_reg  AncestorBlock=xps_library/Memory/software_register  mask(swreg){io_dir=To Processor, io_delay=1, init_val=0, sample_period=1, names=reg, bitwidths=16, bin_pts=0, arith_types=0, sim_port=off, show_format=on}
      mask prompts: io_dir "I/O direction"; io_delay "I/O delay"; init_val "Initial Value"; sample_period "Sample period"; names "Bitfield names [msb...lsb]"; bitwidths "Bitfield widths"; bin_pts "Bitfield binary pts"; arith_types "Bitfield types, ufix=0, fix=1, bool=2"; sim_port "Provide sim input/output?"; show_format "Print format string?"
      mask help: A 32-bit software-accessible register. Can be divided into bitfields of varying widths and types using the fields in the block mask.
      mask init:
      | swreg_init(gcb)
      settings: AttributesFormatString=1output:uf16.0 = 16 bits
      mask TypeOptions io_dir: To Processor | From Processor
      mask Callback io_dir:
      | mask_enables = get_param(gcb, 'MaskEnables');
      | mask_names = get_param(gcb, 'MaskNames');
      | if strcmp(get_param(gcb, 'io_dir'), 'To Processor'),
      |     mask_enables{ismember(mask_names, 'sample_period')} = 'off';
      | else
      |     mask_enables{ismember(mask_names, 'sample_period')} = 'on';
      | end
      | set_param(gcb, 'MaskEnables', mask_enables);
      mask DialogControl ParameterTabVar0 Prompt: Setup
  txctr1_and : xbsIndex_r4/Logical  logical_function=AND  inputs=2  en=off  latency=1  precision=Full  arith_type=Unsigned  n_bits=16  bin_pt=0  align_bp=on  dbl_ovrd=off  block_type=logical
  txctr1_c_pipe : casper_library_delays/pipeline  latency=3
      settings: AttributesFormatString=Latency = %<latency>
  txctr1_ctr : xbsIndex_r4/Counter  cnt_type=Free Running  cnt_to=Inf  operation=Up  start_count=0  cnt_by_val=1  arith_type=Unsigned  n_bits=16  bin_pt=0  load_pin=off  rst=on  en=on  explicit_period=on  period=1  use_behavioral_HDL=on  implementation=Fabric  dbl_ovrd=off  block_type=counter
  txctr1_del : xbsIndex_r4/Delay  rst=off  infoeditControl=Selection of Reset will increase slice count due to use of real FFs and instead of SRLs  en=off  latency=1  reg_retiming=on  dbl_ovrd=off  block_type=delay
      settings: infoedit=Hardware notes: A delay line is a chain, each link of which is an SRL16 or SRL32 followed by a flip-flop.
  txctr1_e_pipe : casper_library_delays/pipeline  latency=3
      settings: AttributesFormatString=Latency = %<latency>
  txctr1_ed : casper_library_misc/edge_detect  edge=Rising  polarity=Active High  x_in=[0 0.08 0.08 0.16 0.16 0.24 0.24 0.32 0.32 0.4]  y_in="[-1 -1  1  1  1  1  1  1  1  1]"  x_out=[0.6 0.68 0.68 0.76 0.76 0.84 0.84 0.92 0.92 1]  y_out="[-1 -1  1  1 -1 -1 -1 -1 -1 -1]"
  txctr1_r_pipe : casper_library_delays/pipeline  latency=3
      settings: AttributesFormatString=Latency = %<latency>
  txctr1_v_pipe : casper_library_delays/pipeline  latency=3
      settings: AttributesFormatString=Latency = %<latency>
  txerrctr0 : Subsystem  Tag=xps:sw_reg  AncestorBlock=xps_library/Memory/software_register  mask(swreg){io_dir=To Processor, io_delay=1, init_val=0, sample_period=1, names=reg, bitwidths=16, bin_pts=0, arith_types=0, sim_port=off, show_format=on}
      mask prompts: io_dir "I/O direction"; io_delay "I/O delay"; init_val "Initial Value"; sample_period "Sample period"; names "Bitfield names [msb...lsb]"; bitwidths "Bitfield widths"; bin_pts "Bitfield binary pts"; arith_types "Bitfield types, ufix=0, fix=1, bool=2"; sim_port "Provide sim input/output?"; show_format "Print format string?"
      mask help: A 32-bit software-accessible register. Can be divided into bitfields of varying widths and types using the fields in the block mask.
      mask init:
      | swreg_init(gcb)
      settings: AttributesFormatString=1output:uf16.0 = 16 bits
      mask TypeOptions io_dir: To Processor | From Processor
      mask Callback io_dir:
      | mask_enables = get_param(gcb, 'MaskEnables');
      | mask_names = get_param(gcb, 'MaskNames');
      | if strcmp(get_param(gcb, 'io_dir'), 'To Processor'),
      |     mask_enables{ismember(mask_names, 'sample_period')} = 'off';
      | else
      |     mask_enables{ismember(mask_names, 'sample_period')} = 'on';
      | end
      | set_param(gcb, 'MaskEnables', mask_enables);
      mask DialogControl ParameterTabVar0 Prompt: Setup
  txerrctr0_b_pipe : casper_library_delays/pipeline  latency=3
      settings: AttributesFormatString=Latency = %<latency>
  txerrctr0_c_pipe : casper_library_delays/pipeline  latency=3
      settings: AttributesFormatString=Latency = %<latency>
  txerrctr0_ctr : xbsIndex_r4/Counter  cnt_type=Free Running  cnt_to=Inf  operation=Up  start_count=0  cnt_by_val=1  arith_type=Unsigned  n_bits=16  bin_pt=0  load_pin=off  rst=on  en=on  explicit_period=on  period=1  use_behavioral_HDL=on  implementation=Fabric  dbl_ovrd=off  block_type=counter
  txerrctr0_del : xbsIndex_r4/Delay  rst=off  infoeditControl=Selection of Reset will increase slice count due to use of real FFs and instead of SRLs  en=off  latency=1  reg_retiming=on  dbl_ovrd=off  block_type=delay
      settings: infoedit=Hardware notes: A delay line is a chain, each link of which is an SRL16 or SRL32 followed by a flip-flop.
  txerrctr0_e_pipe : casper_library_delays/pipeline  latency=3
      settings: AttributesFormatString=Latency = %<latency>
  txerrctr0_errchk : Subsystem  Tag=casper:frame_len_checker  AncestorBlock=casper_library_communications/frame_len_checker  mask{frame_len=100}
      mask prompts: frame_len "Frame length (64-bit words):"
      mask help: Monitors valid, EOF and bad_frame signals in/from a 10Gbe core and outputs an error signal. Can be used to drive an error counter or latched as a flag.
  txerrctr0_errchk_pipe : casper_library_delays/pipeline  latency=3
      settings: AttributesFormatString=Latency = %<latency>
  txerrctr0_nobad : xbsIndex_r4/Constant  const=0  gui_display_data_type=Fixed-point  arith_type=Boolean  n_bits=16  bin_pt=14  preci_type=Single  exp_width=8  frac_width=24  explicit_period=on  period=1  equ=P=C  opselect=C  inp2=PCIN>>17  opr=+  inp1=P  carry=CIN  dbl_ovrd=off  block_type=constant
  txerrctr0_r_pipe : casper_library_delays/pipeline  latency=3
      settings: AttributesFormatString=Latency = %<latency>
  txerrctr0_v_pipe : casper_library_delays/pipeline  latency=3
      settings: AttributesFormatString=Latency = %<latency>
  txerrctr1 : Subsystem  Tag=xps:sw_reg  AncestorBlock=xps_library/Memory/software_register  mask(swreg){io_dir=To Processor, io_delay=1, init_val=0, sample_period=1, names=reg, bitwidths=16, bin_pts=0, arith_types=0, sim_port=off, show_format=on}
      mask prompts: io_dir "I/O direction"; io_delay "I/O delay"; init_val "Initial Value"; sample_period "Sample period"; names "Bitfield names [msb...lsb]"; bitwidths "Bitfield widths"; bin_pts "Bitfield binary pts"; arith_types "Bitfield types, ufix=0, fix=1, bool=2"; sim_port "Provide sim input/output?"; show_format "Print format string?"
      mask help: A 32-bit software-accessible register. Can be divided into bitfields of varying widths and types using the fields in the block mask.
      mask init:
      | swreg_init(gcb)
      settings: AttributesFormatString=1output:uf16.0 = 16 bits
      mask TypeOptions io_dir: To Processor | From Processor
      mask Callback io_dir:
      | mask_enables = get_param(gcb, 'MaskEnables');
      | mask_names = get_param(gcb, 'MaskNames');
      | if strcmp(get_param(gcb, 'io_dir'), 'To Processor'),
      |     mask_enables{ismember(mask_names, 'sample_period')} = 'off';
      | else
      |     mask_enables{ismember(mask_names, 'sample_period')} = 'on';
      | end
      | set_param(gcb, 'MaskEnables', mask_enables);
      mask DialogControl ParameterTabVar0 Prompt: Setup
  txerrctr1_b_pipe : casper_library_delays/pipeline  latency=3
      settings: AttributesFormatString=Latency = %<latency>
  txerrctr1_c_pipe : casper_library_delays/pipeline  latency=3
      settings: AttributesFormatString=Latency = %<latency>
  txerrctr1_ctr : xbsIndex_r4/Counter  cnt_type=Free Running  cnt_to=Inf  operation=Up  start_count=0  cnt_by_val=1  arith_type=Unsigned  n_bits=16  bin_pt=0  load_pin=off  rst=on  en=on  explicit_period=on  period=1  use_behavioral_HDL=on  implementation=Fabric  dbl_ovrd=off  block_type=counter
  txerrctr1_del : xbsIndex_r4/Delay  rst=off  infoeditControl=Selection of Reset will increase slice count due to use of real FFs and instead of SRLs  en=off  latency=1  reg_retiming=on  dbl_ovrd=off  block_type=delay
      settings: infoedit=Hardware notes: A delay line is a chain, each link of which is an SRL16 or SRL32 followed by a flip-flop.
  txerrctr1_e_pipe : casper_library_delays/pipeline  latency=3
      settings: AttributesFormatString=Latency = %<latency>
  txerrctr1_errchk : Subsystem  Tag=casper:frame_len_checker  AncestorBlock=casper_library_communications/frame_len_checker  mask{frame_len=100}
      mask prompts: frame_len "Frame length (64-bit words):"
      mask help: Monitors valid, EOF and bad_frame signals in/from a 10Gbe core and outputs an error signal. Can be used to drive an error counter or latched as a flag.
  txerrctr1_errchk_pipe : casper_library_delays/pipeline  latency=3
      settings: AttributesFormatString=Latency = %<latency>
  txerrctr1_nobad : xbsIndex_r4/Constant  const=0  gui_display_data_type=Fixed-point  arith_type=Boolean  n_bits=16  bin_pt=14  preci_type=Single  exp_width=8  frac_width=24  explicit_period=on  period=1  equ=P=C  opselect=C  inp2=PCIN>>17  opr=+  inp1=P  carry=CIN  dbl_ovrd=off  block_type=constant
  txerrctr1_r_pipe : casper_library_delays/pipeline  latency=3
      settings: AttributesFormatString=Latency = %<latency>
  txerrctr1_v_pipe : casper_library_delays/pipeline  latency=3
      settings: AttributesFormatString=Latency = %<latency>
  txfullctr0 : Subsystem  Tag=xps:sw_reg  AncestorBlock=xps_library/Memory/software_register  mask(swreg){io_dir=To Processor, io_delay=1, init_val=0, sample_period=1, names=reg, bitwidths=16, bin_pts=0, arith_types=0, sim_port=off, show_format=on}
      mask prompts: io_dir "I/O direction"; io_delay "I/O delay"; init_val "Initial Value"; sample_period "Sample period"; names "Bitfield names [msb...lsb]"; bitwidths "Bitfield widths"; bin_pts "Bitfield binary pts"; arith_types "Bitfield types, ufix=0, fix=1, bool=2"; sim_port "Provide sim input/output?"; show_format "Print format string?"
      mask help: A 32-bit software-accessible register. Can be divided into bitfields of varying widths and types using the fields in the block mask.
      mask init:
      | swreg_init(gcb)
      settings: AttributesFormatString=1output:uf16.0 = 16 bits
      mask TypeOptions io_dir: To Processor | From Processor
      mask Callback io_dir:
      | mask_enables = get_param(gcb, 'MaskEnables');
      | mask_names = get_param(gcb, 'MaskNames');
      | if strcmp(get_param(gcb, 'io_dir'), 'To Processor'),
      |     mask_enables{ismember(mask_names, 'sample_period')} = 'off';
      | else
      |     mask_enables{ismember(mask_names, 'sample_period')} = 'on';
      | end
      | set_param(gcb, 'MaskEnables', mask_enables);
      mask DialogControl ParameterTabVar0 Prompt: Setup
  txfullctr0_c_pipe : casper_library_delays/pipeline  latency=3
      settings: AttributesFormatString=Latency = %<latency>
  txfullctr0_ctr : xbsIndex_r4/Counter  cnt_type=Free Running  cnt_to=Inf  operation=Up  start_count=0  cnt_by_val=1  arith_type=Unsigned  n_bits=16  bin_pt=0  load_pin=off  rst=on  en=on  explicit_period=on  period=1  use_behavioral_HDL=on  implementation=Fabric  dbl_ovrd=off  block_type=counter
  txfullctr0_del : xbsIndex_r4/Delay  rst=off  infoeditControl=Selection of Reset will increase slice count due to use of real FFs and instead of SRLs  en=off  latency=1  reg_retiming=on  dbl_ovrd=off  block_type=delay
      settings: infoedit=Hardware notes: A delay line is a chain, each link of which is an SRL16 or SRL32 followed by a flip-flop.
  txfullctr0_r_pipe : casper_library_delays/pipeline  latency=3
      settings: AttributesFormatString=Latency = %<latency>
  txfullctr1 : Subsystem  Tag=xps:sw_reg  AncestorBlock=xps_library/Memory/software_register  mask(swreg){io_dir=To Processor, io_delay=1, init_val=0, sample_period=1, names=reg, bitwidths=16, bin_pts=0, arith_types=0, sim_port=off, show_format=on}
      mask prompts: io_dir "I/O direction"; io_delay "I/O delay"; init_val "Initial Value"; sample_period "Sample period"; names "Bitfield names [msb...lsb]"; bitwidths "Bitfield widths"; bin_pts "Bitfield binary pts"; arith_types "Bitfield types, ufix=0, fix=1, bool=2"; sim_port "Provide sim input/output?"; show_format "Print format string?"
      mask help: A 32-bit software-accessible register. Can be divided into bitfields of varying widths and types using the fields in the block mask.
      mask init:
      | swreg_init(gcb)
      settings: AttributesFormatString=1output:uf16.0 = 16 bits
      mask TypeOptions io_dir: To Processor | From Processor
      mask Callback io_dir:
      | mask_enables = get_param(gcb, 'MaskEnables');
      | mask_names = get_param(gcb, 'MaskNames');
      | if strcmp(get_param(gcb, 'io_dir'), 'To Processor'),
      |     mask_enables{ismember(mask_names, 'sample_period')} = 'off';
      | else
      |     mask_enables{ismember(mask_names, 'sample_period')} = 'on';
      | end
      | set_param(gcb, 'MaskEnables', mask_enables);
      mask DialogControl ParameterTabVar0 Prompt: Setup
  txfullctr1_c_pipe : casper_library_delays/pipeline  latency=3
      settings: AttributesFormatString=Latency = %<latency>
  txfullctr1_ctr : xbsIndex_r4/Counter  cnt_type=Free Running  cnt_to=Inf  operation=Up  start_count=0  cnt_by_val=1  arith_type=Unsigned  n_bits=16  bin_pt=0  load_pin=off  rst=on  en=on  explicit_period=on  period=1  use_behavioral_HDL=on  implementation=Fabric  dbl_ovrd=off  block_type=counter
  txfullctr1_del : xbsIndex_r4/Delay  rst=off  infoeditControl=Selection of Reset will increase slice count due to use of real FFs and instead of SRLs  en=off  latency=1  reg_retiming=on  dbl_ovrd=off  block_type=delay
      settings: infoedit=Hardware notes: A delay line is a chain, each link of which is an SRL16 or SRL32 followed by a flip-flop.
  txfullctr1_r_pipe : casper_library_delays/pipeline  latency=3
      settings: AttributesFormatString=Latency = %<latency>
  txofctr0 : Subsystem  Tag=xps:sw_reg  AncestorBlock=xps_library/Memory/software_register  mask(swreg){io_dir=To Processor, io_delay=1, init_val=0, sample_period=1, names=reg, bitwidths=16, bin_pts=0, arith_types=0, sim_port=off, show_format=on}
      mask prompts: io_dir "I/O direction"; io_delay "I/O delay"; init_val "Initial Value"; sample_period "Sample period"; names "Bitfield names [msb...lsb]"; bitwidths "Bitfield widths"; bin_pts "Bitfield binary pts"; arith_types "Bitfield types, ufix=0, fix=1, bool=2"; sim_port "Provide sim input/output?"; show_format "Print format string?"
      mask help: A 32-bit software-accessible register. Can be divided into bitfields of varying widths and types using the fields in the block mask.
      mask init:
      | swreg_init(gcb)
      settings: AttributesFormatString=1output:uf16.0 = 16 bits
      mask TypeOptions io_dir: To Processor | From Processor
      mask Callback io_dir:
      | mask_enables = get_param(gcb, 'MaskEnables');
      | mask_names = get_param(gcb, 'MaskNames');
      | if strcmp(get_param(gcb, 'io_dir'), 'To Processor'),
      |     mask_enables{ismember(mask_names, 'sample_period')} = 'off';
      | else
      |     mask_enables{ismember(mask_names, 'sample_period')} = 'on';
      | end
      | set_param(gcb, 'MaskEnables', mask_enables);
      mask DialogControl ParameterTabVar0 Prompt: Setup
  txofctr0_c_pipe : casper_library_delays/pipeline  latency=3
      settings: AttributesFormatString=Latency = %<latency>
  txofctr0_ctr : xbsIndex_r4/Counter  cnt_type=Free Running  cnt_to=Inf  operation=Up  start_count=0  cnt_by_val=1  arith_type=Unsigned  n_bits=16  bin_pt=0  load_pin=off  rst=on  en=on  explicit_period=on  period=1  use_behavioral_HDL=on  implementation=Fabric  dbl_ovrd=off  block_type=counter
  txofctr0_del : xbsIndex_r4/Delay  rst=off  infoeditControl=Selection of Reset will increase slice count due to use of real FFs and instead of SRLs  en=off  latency=1  reg_retiming=on  dbl_ovrd=off  block_type=delay
      settings: infoedit=Hardware notes: A delay line is a chain, each link of which is an SRL16 or SRL32 followed by a flip-flop.
  txofctr0_r_pipe : casper_library_delays/pipeline  latency=3
      settings: AttributesFormatString=Latency = %<latency>
  txofctr1 : Subsystem  Tag=xps:sw_reg  AncestorBlock=xps_library/Memory/software_register  mask(swreg){io_dir=To Processor, io_delay=1, init_val=0, sample_period=1, names=reg, bitwidths=16, bin_pts=0, arith_types=0, sim_port=off, show_format=on}
      mask prompts: io_dir "I/O direction"; io_delay "I/O delay"; init_val "Initial Value"; sample_period "Sample period"; names "Bitfield names [msb...lsb]"; bitwidths "Bitfield widths"; bin_pts "Bitfield binary pts"; arith_types "Bitfield types, ufix=0, fix=1, bool=2"; sim_port "Provide sim input/output?"; show_format "Print format string?"
      mask help: A 32-bit software-accessible register. Can be divided into bitfields of varying widths and types using the fields in the block mask.
      mask init:
      | swreg_init(gcb)
      settings: AttributesFormatString=1output:uf16.0 = 16 bits
      mask TypeOptions io_dir: To Processor | From Processor
      mask Callback io_dir:
      | mask_enables = get_param(gcb, 'MaskEnables');
      | mask_names = get_param(gcb, 'MaskNames');
      | if strcmp(get_param(gcb, 'io_dir'), 'To Processor'),
      |     mask_enables{ismember(mask_names, 'sample_period')} = 'off';
      | else
      |     mask_enables{ismember(mask_names, 'sample_period')} = 'on';
      | end
      | set_param(gcb, 'MaskEnables', mask_enables);
      mask DialogControl ParameterTabVar0 Prompt: Setup
  txofctr1_c_pipe : casper_library_delays/pipeline  latency=3
      settings: AttributesFormatString=Latency = %<latency>
  txofctr1_ctr : xbsIndex_r4/Counter  cnt_type=Free Running  cnt_to=Inf  operation=Up  start_count=0  cnt_by_val=1  arith_type=Unsigned  n_bits=16  bin_pt=0  load_pin=off  rst=on  en=on  explicit_period=on  period=1  use_behavioral_HDL=on  implementation=Fabric  dbl_ovrd=off  block_type=counter
  txofctr1_del : xbsIndex_r4/Delay  rst=off  infoeditControl=Selection of Reset will increase slice count due to use of real FFs and instead of SRLs  en=off  latency=1  reg_retiming=on  dbl_ovrd=off  block_type=delay
      settings: infoedit=Hardware notes: A delay line is a chain, each link of which is an SRL16 or SRL32 followed by a flip-flop.
  txofctr1_r_pipe : casper_library_delays/pipeline  latency=3
      settings: AttributesFormatString=Latency = %<latency>
  txvldctr0 : Subsystem  Tag=xps:sw_reg  AncestorBlock=xps_library/Memory/software_register  mask(swreg){io_dir=To Processor, io_delay=1, init_val=0, sample_period=1, names=reg, bitwidths=16, bin_pts=0, arith_types=0, sim_port=off, show_format=on}
      mask prompts: io_dir "I/O direction"; io_delay "I/O delay"; init_val "Initial Value"; sample_period "Sample period"; names "Bitfield names [msb...lsb]"; bitwidths "Bitfield widths"; bin_pts "Bitfield binary pts"; arith_types "Bitfield types, ufix=0, fix=1, bool=2"; sim_port "Provide sim input/output?"; show_format "Print format string?"
      mask help: A 32-bit software-accessible register. Can be divided into bitfields of varying widths and types using the fields in the block mask.
      mask init:
      | swreg_init(gcb)
      settings: AttributesFormatString=1output:uf16.0 = 16 bits
      mask TypeOptions io_dir: To Processor | From Processor
      mask Callback io_dir:
      | mask_enables = get_param(gcb, 'MaskEnables');
      | mask_names = get_param(gcb, 'MaskNames');
      | if strcmp(get_param(gcb, 'io_dir'), 'To Processor'),
      |     mask_enables{ismember(mask_names, 'sample_period')} = 'off';
      | else
      |     mask_enables{ismember(mask_names, 'sample_period')} = 'on';
      | end
      | set_param(gcb, 'MaskEnables', mask_enables);
      mask DialogControl ParameterTabVar0 Prompt: Setup
  txvldctr0_c_pipe : casper_library_delays/pipeline  latency=3
      settings: AttributesFormatString=Latency = %<latency>
  txvldctr0_ctr : xbsIndex_r4/Counter  cnt_type=Free Running  cnt_to=Inf  operation=Up  start_count=0  cnt_by_val=1  arith_type=Unsigned  n_bits=16  bin_pt=0  load_pin=off  rst=on  en=on  explicit_period=on  period=1  use_behavioral_HDL=on  implementation=Fabric  dbl_ovrd=off  block_type=counter
  txvldctr0_del : xbsIndex_r4/Delay  rst=off  infoeditControl=Selection of Reset will increase slice count due to use of real FFs and instead of SRLs  en=off  latency=1  reg_retiming=on  dbl_ovrd=off  block_type=delay
      settings: infoedit=Hardware notes: A delay line is a chain, each link of which is an SRL16 or SRL32 followed by a flip-flop.
  txvldctr0_r_pipe : casper_library_delays/pipeline  latency=3
      settings: AttributesFormatString=Latency = %<latency>
  txvldctr1 : Subsystem  Tag=xps:sw_reg  AncestorBlock=xps_library/Memory/software_register  mask(swreg){io_dir=To Processor, io_delay=1, init_val=0, sample_period=1, names=reg, bitwidths=16, bin_pts=0, arith_types=0, sim_port=off, show_format=on}
      mask prompts: io_dir "I/O direction"; io_delay "I/O delay"; init_val "Initial Value"; sample_period "Sample period"; names "Bitfield names [msb...lsb]"; bitwidths "Bitfield widths"; bin_pts "Bitfield binary pts"; arith_types "Bitfield types, ufix=0, fix=1, bool=2"; sim_port "Provide sim input/output?"; show_format "Print format string?"
      mask help: A 32-bit software-accessible register. Can be divided into bitfields of varying widths and types using the fields in the block mask.
      mask init:
      | swreg_init(gcb)
      settings: AttributesFormatString=1output:uf16.0 = 16 bits
      mask TypeOptions io_dir: To Processor | From Processor
      mask Callback io_dir:
      | mask_enables = get_param(gcb, 'MaskEnables');
      | mask_names = get_param(gcb, 'MaskNames');
      | if strcmp(get_param(gcb, 'io_dir'), 'To Processor'),
      |     mask_enables{ismember(mask_names, 'sample_period')} = 'off';
      | else
      |     mask_enables{ismember(mask_names, 'sample_period')} = 'on';
      | end
      | set_param(gcb, 'MaskEnables', mask_enables);
      mask DialogControl ParameterTabVar0 Prompt: Setup
  txvldctr1_c_pipe : casper_library_delays/pipeline  latency=3
      settings: AttributesFormatString=Latency = %<latency>
  txvldctr1_ctr : xbsIndex_r4/Counter  cnt_type=Free Running  cnt_to=Inf  operation=Up  start_count=0  cnt_by_val=1  arith_type=Unsigned  n_bits=16  bin_pt=0  load_pin=off  rst=on  en=on  explicit_period=on  period=1  use_behavioral_HDL=on  implementation=Fabric  dbl_ovrd=off  block_type=counter
  txvldctr1_del : xbsIndex_r4/Delay  rst=off  infoeditControl=Selection of Reset will increase slice count due to use of real FFs and instead of SRLs  en=off  latency=1  reg_retiming=on  dbl_ovrd=off  block_type=delay
      settings: infoedit=Hardware notes: A delay line is a chain, each link of which is an SRL16 or SRL32 followed by a flip-flop.
  txvldctr1_r_pipe : casper_library_delays/pipeline  latency=3
      settings: AttributesFormatString=Latency = %<latency>
  led_up0 : Outport
  led_tx0 : Outport  Port=2
  tx_afull0 : Outport  Port=3
  tx_overflow0 : Outport  Port=4
  led_rx0 : Outport  Port=5
  rx_valid0 : Outport  Port=6
  rx_data0 : Outport  Port=7
  rx_source_ip0 : Outport  Port=8
  rx_source_port0 : Outport  Port=9
  rx_dest_ip0 : Outport  Port=10
  rx_dest_port0 : Outport  Port=11
  rx_end_of_frame0 : Outport  Port=12
  rx_bad_frame0 : Outport  Port=13
  rx_overrun0 : Outport  Port=14
  led_up1 : Outport  Port=15
  led_tx1 : Outport  Port=16
  tx_afull1 : Outport  Port=17
  tx_overflow1 : Outport  Port=18
  led_rx1 : Outport  Port=19
  rx_valid1 : Outport  Port=20
  rx_data1 : Outport  Port=21
  rx_source_ip1 : Outport  Port=22
  rx_source_port1 : Outport  Port=23
  rx_dest_ip1 : Outport  Port=24
  rx_dest_port1 : Outport  Port=25
  rx_end_of_frame1 : Outport  Port=26
  rx_bad_frame1 : Outport  Port=27
  rx_overrun1 : Outport  Port=28
  wires:
  led_up0_const/1 -> skarab_fgbe_forty_gbe_led_up0/1
  skarab_fgbe_forty_gbe_led_up0/1 -> led_up0_pipe/1
  led_up0_pipe/1 -> led_up0/1
  led_tx0_const/1 -> skarab_fgbe_forty_gbe_led_tx0/1
  skarab_fgbe_forty_gbe_led_tx0/1 -> led_tx0_pipe/1
  led_tx0_pipe/1 -> led_tx0/1
  tx_afull0_const/1 -> skarab_fgbe_forty_gbe_tx_afull0/1
  skarab_fgbe_forty_gbe_tx_afull0/1 -> tx_afull0_pipe/1
  tx_afull0_pipe/1 -> tx_afull0/1, txfullctr0_ctr/2
  tx_overflow0_const/1 -> skarab_fgbe_forty_gbe_tx_overflow0/1
  skarab_fgbe_forty_gbe_tx_overflow0/1 -> tx_overflow0_pipe/1
  tx_overflow0_pipe/1 -> tx_overflow0/1, txofctr0_ctr/2
  led_rx0_const/1 -> skarab_fgbe_forty_gbe_led_rx0/1
  skarab_fgbe_forty_gbe_led_rx0/1 -> led_rx0_pipe/1
  led_rx0_pipe/1 -> led_rx0/1
  rx_valid0_const/1 -> skarab_fgbe_forty_gbe_rx_valid0/1
  skarab_fgbe_forty_gbe_rx_valid0/1 -> rx_valid0_pipe/1
  rx_valid0_pipe/1 -> rx_valid0/1, rx_vld_bus0/1(bus_in)
  rx_data0_const/1 -> skarab_fgbe_forty_gbe_rx_data0/1
  skarab_fgbe_forty_gbe_rx_data0/1 -> rx_data0_pipe/1
  rx_data0_pipe/1 -> rx_data0/1
  rx_source_ip0_const/1 -> skarab_fgbe_forty_gbe_rx_source_ip0/1
  skarab_fgbe_forty_gbe_rx_source_ip0/1 -> rx_source_ip0_pipe/1
  rx_source_ip0_pipe/1 -> rx_source_ip0/1
  rx_source_port0_const/1 -> skarab_fgbe_forty_gbe_rx_source_port0/1
  skarab_fgbe_forty_gbe_rx_source_port0/1 -> rx_source_port0_pipe/1
  rx_source_port0_pipe/1 -> rx_source_port0/1
  rx_dest_ip0_const/1 -> skarab_fgbe_forty_gbe_rx_dest_ip0/1
  skarab_fgbe_forty_gbe_rx_dest_ip0/1 -> rx_dest_ip0_pipe/1
  rx_dest_ip0_pipe/1 -> rx_dest_ip0/1
  rx_dest_port0_const/1 -> skarab_fgbe_forty_gbe_rx_dest_port0/1
  skarab_fgbe_forty_gbe_rx_dest_port0/1 -> rx_dest_port0_pipe/1
  rx_dest_port0_pipe/1 -> rx_dest_port0/1
  rx_end_of_frame0_const/1 -> skarab_fgbe_forty_gbe_rx_end_of_frame0/1
  skarab_fgbe_forty_gbe_rx_end_of_frame0/1 -> rx_end_of_frame0_pipe/1
  rx_end_of_frame0_pipe/1 -> rx_end_of_frame0/1, rx_eof0_pipe/1, rxeofctr0_ctr/2
  rx_bad_frame0_const/1 -> skarab_fgbe_forty_gbe_rx_bad_frame0/1
  skarab_fgbe_forty_gbe_rx_bad_frame0/1 -> rx_bad_frame0_pipe/1
  rx_bad_frame0_pipe/1 -> rx_bad_frame0/1, rxbadctr0_ctr/2
  rx_overrun0_const/1 -> skarab_fgbe_forty_gbe_rx_overrun0/1
  skarab_fgbe_forty_gbe_rx_overrun0/1 -> rx_overrun0_pipe/1
  rx_overrun0_pipe/1 -> rx_overrun0/1, rxofctr0_ctr/2
  rx_vld_bus0/1(msb_out4) -> rx_vld_or0/1
  rx_vld_bus0/2(out3) -> rx_vld_or0/2
  rx_vld_bus0/3(out2) -> rx_vld_or0/3
  rx_vld_bus0/4(lsb_out1) -> rx_vld_or0/4
  rx_vld_or0/1 -> rx_vld_or_out_0_pipe/1(d)
  led_up1_const/1 -> skarab_fgbe_forty_gbe_led_up1/1
  skarab_fgbe_forty_gbe_led_up1/1 -> led_up1_pipe/1
  led_up1_pipe/1 -> led_up1/1
  led_tx1_const/1 -> skarab_fgbe_forty_gbe_led_tx1/1
  skarab_fgbe_forty_gbe_led_tx1/1 -> led_tx1_pipe/1
  led_tx1_pipe/1 -> led_tx1/1
  tx_afull1_const/1 -> skarab_fgbe_forty_gbe_tx_afull1/1
  skarab_fgbe_forty_gbe_tx_afull1/1 -> tx_afull1_pipe/1
  tx_afull1_pipe/1 -> tx_afull1/1, txfullctr1_ctr/2
  tx_overflow1_const/1 -> skarab_fgbe_forty_gbe_tx_overflow1/1
  skarab_fgbe_forty_gbe_tx_overflow1/1 -> tx_overflow1_pipe/1
  tx_overflow1_pipe/1 -> tx_overflow1/1, txofctr1_ctr/2
  led_rx1_const/1 -> skarab_fgbe_forty_gbe_led_rx1/1
  skarab_fgbe_forty_gbe_led_rx1/1 -> led_rx1_pipe/1
  led_rx1_pipe/1 -> led_rx1/1
  rx_valid1_const/1 -> skarab_fgbe_forty_gbe_rx_valid1/1
  skarab_fgbe_forty_gbe_rx_valid1/1 -> rx_valid1_pipe/1
  rx_valid1_pipe/1 -> rx_valid1/1, rx_vld_bus1/1(bus_in)
  rx_data1_const/1 -> skarab_fgbe_forty_gbe_rx_data1/1
  skarab_fgbe_forty_gbe_rx_data1/1 -> rx_data1_pipe/1
  rx_data1_pipe/1 -> rx_data1/1
  rx_source_ip1_const/1 -> skarab_fgbe_forty_gbe_rx_source_ip1/1
  skarab_fgbe_forty_gbe_rx_source_ip1/1 -> rx_source_ip1_pipe/1
  rx_source_ip1_pipe/1 -> rx_source_ip1/1
  rx_source_port1_const/1 -> skarab_fgbe_forty_gbe_rx_source_port1/1
  skarab_fgbe_forty_gbe_rx_source_port1/1 -> rx_source_port1_pipe/1
  rx_source_port1_pipe/1 -> rx_source_port1/1
  rx_dest_ip1_const/1 -> skarab_fgbe_forty_gbe_rx_dest_ip1/1
  skarab_fgbe_forty_gbe_rx_dest_ip1/1 -> rx_dest_ip1_pipe/1
  rx_dest_ip1_pipe/1 -> rx_dest_ip1/1
  rx_dest_port1_const/1 -> skarab_fgbe_forty_gbe_rx_dest_port1/1
  skarab_fgbe_forty_gbe_rx_dest_port1/1 -> rx_dest_port1_pipe/1
  rx_dest_port1_pipe/1 -> rx_dest_port1/1
  rx_end_of_frame1_const/1 -> skarab_fgbe_forty_gbe_rx_end_of_frame1/1
  skarab_fgbe_forty_gbe_rx_end_of_frame1/1 -> rx_end_of_frame1_pipe/1
  rx_end_of_frame1_pipe/1 -> rx_end_of_frame1/1, rx_eof1_pipe/1(d), rxeofctr1_ctr/2
  rx_bad_frame1_const/1 -> skarab_fgbe_forty_gbe_rx_bad_frame1/1
  skarab_fgbe_forty_gbe_rx_bad_frame1/1 -> rx_bad_frame1_pipe/1
  rx_bad_frame1_pipe/1 -> rx_bad_frame1/1, rxbadctr1_ctr/2
  rx_overrun1_const/1 -> skarab_fgbe_forty_gbe_rx_overrun1/1
  skarab_fgbe_forty_gbe_rx_overrun1/1 -> rx_overrun1_pipe/1
  rx_overrun1_pipe/1 -> rx_overrun1/1, rxofctr1_ctr/2
  rx_vld_bus1/1(msb_out4) -> rx_vld_or1/1
  rx_vld_bus1/2(out3) -> rx_vld_or1/2
  rx_vld_bus1/3(out2) -> rx_vld_or1/3
  rx_vld_bus1/4(lsb_out1) -> rx_vld_or1/4
  rx_vld_or1/1 -> rx_vld_or_out_1_pipe/1(d)
  tx_valid0/1 -> tx_valid0_apipe/1, txctr0_e_pipe/1, txerrctr0_v_pipe/1
  tx_valid0_apipe/1 -> tx_valid0_assert/1
  tx_valid0_assert/1 -> tx_valid0_pipe/1
  tx_valid0_pipe/1 -> skarab_fgbe_forty_gbe_tx_valid0/1, txvldctr0_ctr/2
  skarab_fgbe_forty_gbe_tx_valid0/1 -> -6_term/1
  tx_end_of_frame0/1 -> tx_end_of_frame0_apipe/1, txctr0_v_pipe/1, txerrctr0_e_pipe/1
  tx_end_of_frame0_apipe/1 -> tx_end_of_frame0_assert/1
  tx_end_of_frame0_assert/1 -> tx_end_of_frame0_pipe/1
  tx_end_of_frame0_pipe/1 -> skarab_fgbe_forty_gbe_tx_end_of_frame0/1
  skarab_fgbe_forty_gbe_tx_end_of_frame0/1 -> -5_term/1
  tx_data0/1 -> tx_data0_apipe/1
  tx_data0_apipe/1 -> tx_data0_assert/1
  tx_data0_assert/1 -> tx_data0_pipe/1
  tx_data0_pipe/1 -> skarab_fgbe_forty_gbe_tx_data0/1
  skarab_fgbe_forty_gbe_tx_data0/1 -> -4_term/1
  tx_dest_ip0/1 -> tx_dest_ip0_apipe/1
  tx_dest_ip0_apipe/1 -> tx_dest_ip0_assert/1
  tx_dest_ip0_assert/1 -> tx_dest_ip0_pipe/1
  tx_dest_ip0_pipe/1 -> skarab_fgbe_forty_gbe_tx_dest_ip0/1
  skarab_fgbe_forty_gbe_tx_dest_ip0/1 -> -3_term/1
  tx_dest_port0/1 -> tx_dest_port0_apipe/1
  tx_dest_port0_apipe/1 -> tx_dest_port0_assert/1
  tx_dest_port0_assert/1 -> tx_dest_port0_pipe/1
  tx_dest_port0_pipe/1 -> skarab_fgbe_forty_gbe_tx_dest_port0/1
  skarab_fgbe_forty_gbe_tx_dest_port0/1 -> -2_term/1
  rx_ack0/1 -> rx_ack0_apipe/1
  rx_ack0_apipe/1 -> rx_ack0_assert/1
  rx_ack0_assert/1 -> rx_ack0_pipe/1
  rx_ack0_pipe/1 -> skarab_fgbe_forty_gbe_rx_ack0/1
  skarab_fgbe_forty_gbe_rx_ack0/1 -> -1_term/1
  rx_overrun_ack0/1 -> rx_overrun_ack0_apipe/1
  rx_overrun_ack0_apipe/1 -> rx_overrun_ack0_assert/1
  rx_overrun_ack0_assert/1 -> rx_overrun_ack0_pipe/1
  rx_overrun_ack0_pipe/1 -> skarab_fgbe_forty_gbe_rx_overrun_ack0/1
  skarab_fgbe_forty_gbe_rx_overrun_ack0/1 -> 0_term/1
  tx_valid1/1 -> tx_valid1_apipe/1, txctr1_e_pipe/1, txerrctr1_v_pipe/1
  tx_valid1_apipe/1 -> tx_valid1_assert/1
  tx_valid1_assert/1 -> tx_valid1_pipe/1
  tx_valid1_pipe/1 -> skarab_fgbe_forty_gbe_tx_valid1/1, txvldctr1_ctr/2
  skarab_fgbe_forty_gbe_tx_valid1/1 -> 1_term/1
  tx_end_of_frame1/1 -> tx_end_of_frame1_apipe/1, txctr1_v_pipe/1, txerrctr1_e_pipe/1
  tx_end_of_frame1_apipe/1 -> tx_end_of_frame1_assert/1
  tx_end_of_frame1_assert/1 -> tx_end_of_frame1_pipe/1
  tx_end_of_frame1_pipe/1 -> skarab_fgbe_forty_gbe_tx_end_of_frame1/1
  skarab_fgbe_forty_gbe_tx_end_of_frame1/1 -> 2_term/1
  tx_data1/1 -> tx_data1_apipe/1
  tx_data1_apipe/1 -> tx_data1_assert/1
  tx_data1_assert/1 -> tx_data1_pipe/1
  tx_data1_pipe/1 -> skarab_fgbe_forty_gbe_tx_data1/1
  skarab_fgbe_forty_gbe_tx_data1/1 -> 3_term/1
  tx_dest_ip1/1 -> tx_dest_ip1_apipe/1
  tx_dest_ip1_apipe/1 -> tx_dest_ip1_assert/1
  tx_dest_ip1_assert/1 -> tx_dest_ip1_pipe/1
  tx_dest_ip1_pipe/1 -> skarab_fgbe_forty_gbe_tx_dest_ip1/1
  skarab_fgbe_forty_gbe_tx_dest_ip1/1 -> 4_term/1
  tx_dest_port1/1 -> tx_dest_port1_apipe/1
  tx_dest_port1_apipe/1 -> tx_dest_port1_assert/1
  tx_dest_port1_assert/1 -> tx_dest_port1_pipe/1
  tx_dest_port1_pipe/1 -> skarab_fgbe_forty_gbe_tx_dest_port1/1
  skarab_fgbe_forty_gbe_tx_dest_port1/1 -> 5_term/1
  rx_ack1/1 -> rx_ack1_apipe/1
  rx_ack1_apipe/1 -> rx_ack1_assert/1
  rx_ack1_assert/1 -> rx_ack1_pipe/1
  rx_ack1_pipe/1 -> skarab_fgbe_forty_gbe_rx_ack1/1
  skarab_fgbe_forty_gbe_rx_ack1/1 -> 6_term/1
  rx_overrun_ack1/1 -> rx_overrun_ack1_apipe/1
  rx_overrun_ack1_apipe/1 -> rx_overrun_ack1_assert/1
  rx_overrun_ack1_assert/1 -> rx_overrun_ack1_pipe/1
  rx_overrun_ack1_pipe/1 -> skarab_fgbe_forty_gbe_rx_overrun_ack1/1
  skarab_fgbe_forty_gbe_rx_overrun_ack1/1 -> 7_term/1
  debug_rst/1 -> term1/1, txctr0_del/1, txerrctr0_del/1, txofctr0_del/1, txfullctr0_del/1, txvldctr0_del/1, rxctr0_del/1, rxerrctr0_del/1, rxofctr0_del/1, rxbadctr0_del/1, rxvldctr0_del/1, rxeofctr0_del/1, txctr1_del/1, txerrctr1_del/1, txofctr1_del/1, txfullctr1_del/1, txvldctr1_del/1, rxctr1_del/1, rxerrctr1_del/1, rxofctr1_del/1, rxbadctr1_del/1, rxvldctr1_del/1, rxeofctr1_del/1
  txctr0_v_pipe/1 -> txctr0_and/1
  txctr0_e_pipe/1 -> txctr0_and/2
  txctr0_and/1 -> txctr0_ed/1
  txctr0_del/1 -> txctr0_r_pipe/1
  txctr0_r_pipe/1 -> txctr0_ctr/1
  txctr0_ed/1 -> txctr0_ctr/2
  txctr0_ctr/1 -> txctr0_c_pipe/1
  txctr0_c_pipe/1 -> txctr0/1(out_reg)
  txerrctr0_v_pipe/1 -> txerrctr0_errchk/1(valid)
  txerrctr0_e_pipe/1 -> txerrctr0_errchk/2(eof)
  txerrctr0_nobad/1 -> txerrctr0_b_pipe/1
  txerrctr0_b_pipe/1 -> txerrctr0_errchk/3(bad_frame)
  txerrctr0_del/1 -> txerrctr0_r_pipe/1
  txerrctr0_r_pipe/1 -> txerrctr0_ctr/1
  txerrctr0_errchk/1(frame_len_error) -> txerrctr0_errchk_pipe/1
  txerrctr0_errchk_pipe/1 -> txerrctr0_ctr/2
  txerrctr0_ctr/1 -> txerrctr0_c_pipe/1
  txerrctr0_c_pipe/1 -> txerrctr0/1(out_reg)
  txofctr0_del/1 -> txofctr0_r_pipe/1
  txofctr0_r_pipe/1 -> txofctr0_ctr/1
  txofctr0_ctr/1 -> txofctr0_c_pipe/1
  txofctr0_c_pipe/1 -> txofctr0/1(out_reg)
  txfullctr0_del/1 -> txfullctr0_r_pipe/1
  txfullctr0_r_pipe/1 -> txfullctr0_ctr/1
  txfullctr0_ctr/1 -> txfullctr0_c_pipe/1
  txfullctr0_c_pipe/1 -> txfullctr0/1(out_reg)
  txvldctr0_del/1 -> txvldctr0_r_pipe/1
  txvldctr0_r_pipe/1 -> txvldctr0_ctr/1
  txvldctr0_ctr/1 -> txvldctr0_c_pipe/1
  txvldctr0_c_pipe/1 -> txvldctr0/1(out_reg)
  rx_eof0_pipe/1 -> rxctr0_v_pipe/1, rxerrctr0_e_pipe/1
  rxctr0_v_pipe/1 -> rxctr0_and/1
  rx_vld_or_out_0_pipe/1(q) -> rxctr0_e_pipe/1, rxerrctr0_v_pipe/1, rxvldctr0_ctr/2
  rxctr0_e_pipe/1 -> rxctr0_and/2
  rxctr0_and/1 -> rxctr0_ed/1
  rxctr0_del/1 -> rxctr0_r_pipe/1
  rxctr0_r_pipe/1 -> rxctr0_ctr/1
  rxctr0_ed/1 -> rxctr0_ctr/2
  rxctr0_ctr/1 -> rxctr0_c_pipe/1
  rxctr0_c_pipe/1 -> rxctr0/1(out_reg)
  rxerrctr0_v_pipe/1 -> rxerrctr0_errchk/1(valid)
  rxerrctr0_e_pipe/1 -> rxerrctr0_errchk/2(eof)
  rxerrctr0_nobad/1 -> rxerrctr0_b_pipe/1
  rxerrctr0_b_pipe/1 -> rxerrctr0_errchk/3(bad_frame)
  rxerrctr0_del/1 -> rxerrctr0_r_pipe/1
  rxerrctr0_r_pipe/1 -> rxerrctr0_ctr/1
  rxerrctr0_errchk/1(frame_len_error) -> rxerrctr0_errchk_pipe/1
  rxerrctr0_errchk_pipe/1 -> rxerrctr0_ctr/2
  rxerrctr0_ctr/1 -> rxerrctr0_c_pipe/1
  rxerrctr0_c_pipe/1 -> rxerrctr0/1(out_reg)
  rxofctr0_del/1 -> rxofctr0_r_pipe/1
  rxofctr0_r_pipe/1 -> rxofctr0_ctr/1
  rxofctr0_ctr/1 -> rxofctr0_c_pipe/1
  rxofctr0_c_pipe/1 -> rxofctr0/1(out_reg)
  rxbadctr0_del/1 -> rxbadctr0_r_pipe/1
  rxbadctr0_r_pipe/1 -> rxbadctr0_ctr/1
  rxbadctr0_ctr/1 -> rxbadctr0_c_pipe/1
  rxbadctr0_c_pipe/1 -> rxbadctr0/1(out_reg)
  rxvldctr0_del/1 -> rxvldctr0_r_pipe/1
  rxvldctr0_r_pipe/1 -> rxvldctr0_ctr/1
  rxvldctr0_ctr/1 -> rxvldctr0_c_pipe/1
  rxvldctr0_c_pipe/1 -> rxvldctr0/1(out_reg)
  rxeofctr0_del/1 -> rxeofctr0_r_pipe/1
  rxeofctr0_r_pipe/1 -> rxeofctr0_ctr/1
  rxeofctr0_ctr/1 -> rxeofctr0_c_pipe/1
  rxeofctr0_c_pipe/1 -> rxeofctr0/1(out_reg)
  txctr1_v_pipe/1 -> txctr1_and/1
  txctr1_e_pipe/1 -> txctr1_and/2
  txctr1_and/1 -> txctr1_ed/1
  txctr1_del/1 -> txctr1_r_pipe/1
  txctr1_r_pipe/1 -> txctr1_ctr/1
  txctr1_ed/1 -> txctr1_ctr/2
  txctr1_ctr/1 -> txctr1_c_pipe/1
  txctr1_c_pipe/1 -> txctr1/1(out_reg)
  txerrctr1_v_pipe/1 -> txerrctr1_errchk/1(valid)
  txerrctr1_e_pipe/1 -> txerrctr1_errchk/2(eof)
  txerrctr1_nobad/1 -> txerrctr1_b_pipe/1
  txerrctr1_b_pipe/1 -> txerrctr1_errchk/3(bad_frame)
  txerrctr1_del/1 -> txerrctr1_r_pipe/1
  txerrctr1_r_pipe/1 -> txerrctr1_ctr/1
  txerrctr1_errchk/1(frame_len_error) -> txerrctr1_errchk_pipe/1
  txerrctr1_errchk_pipe/1 -> txerrctr1_ctr/2
  txerrctr1_ctr/1 -> txerrctr1_c_pipe/1
  txerrctr1_c_pipe/1 -> txerrctr1/1(out_reg)
  txofctr1_del/1 -> txofctr1_r_pipe/1
  txofctr1_r_pipe/1 -> txofctr1_ctr/1
  txofctr1_ctr/1 -> txofctr1_c_pipe/1
  txofctr1_c_pipe/1 -> txofctr1/1(out_reg)
  txfullctr1_del/1 -> txfullctr1_r_pipe/1
  txfullctr1_r_pipe/1 -> txfullctr1_ctr/1
  txfullctr1_ctr/1 -> txfullctr1_c_pipe/1
  txfullctr1_c_pipe/1 -> txfullctr1/1(out_reg)
  txvldctr1_del/1 -> txvldctr1_r_pipe/1
  txvldctr1_r_pipe/1 -> txvldctr1_ctr/1
  txvldctr1_ctr/1 -> txvldctr1_c_pipe/1
  txvldctr1_c_pipe/1 -> txvldctr1/1(out_reg)
  rx_eof1_pipe/1(q) -> rxctr1_v_pipe/1, rxerrctr1_e_pipe/1
  rxctr1_v_pipe/1 -> rxctr1_and/1
  rx_vld_or_out_1_pipe/1(q) -> rxctr1_e_pipe/1, rxerrctr1_v_pipe/1, rxvldctr1_ctr/2
  rxctr1_e_pipe/1 -> rxctr1_and/2
  rxctr1_and/1 -> rxctr1_ed/1
  rxctr1_del/1 -> rxctr1_r_pipe/1
  rxctr1_r_pipe/1 -> rxctr1_ctr/1
  rxctr1_ed/1 -> rxctr1_ctr/2
  rxctr1_ctr/1 -> rxctr1_c_pipe/1
  rxctr1_c_pipe/1 -> rxctr1/1(out_reg)
  rxerrctr1_v_pipe/1 -> rxerrctr1_errchk/1(valid)
  rxerrctr1_e_pipe/1 -> rxerrctr1_errchk/2(eof)
  rxerrctr1_nobad/1 -> rxerrctr1_b_pipe/1
  rxerrctr1_b_pipe/1 -> rxerrctr1_errchk/3(bad_frame)
  rxerrctr1_del/1 -> rxerrctr1_r_pipe/1
  rxerrctr1_r_pipe/1 -> rxerrctr1_ctr/1
  rxerrctr1_errchk/1(frame_len_error) -> rxerrctr1_errchk_pipe/1
  rxerrctr1_errchk_pipe/1 -> rxerrctr1_ctr/2
  rxerrctr1_ctr/1 -> rxerrctr1_c_pipe/1
  rxerrctr1_c_pipe/1 -> rxerrctr1/1(out_reg)
  rxofctr1_del/1 -> rxofctr1_r_pipe/1
  rxofctr1_r_pipe/1 -> rxofctr1_ctr/1
  rxofctr1_ctr/1 -> rxofctr1_c_pipe/1
  rxofctr1_c_pipe/1 -> rxofctr1/1(out_reg)
  rxbadctr1_del/1 -> rxbadctr1_r_pipe/1
  rxbadctr1_r_pipe/1 -> rxbadctr1_ctr/1
  rxbadctr1_ctr/1 -> rxbadctr1_c_pipe/1
  rxbadctr1_c_pipe/1 -> rxbadctr1/1(out_reg)
  rxvldctr1_del/1 -> rxvldctr1_r_pipe/1
  rxvldctr1_r_pipe/1 -> rxvldctr1_ctr/1
  rxvldctr1_ctr/1 -> rxvldctr1_c_pipe/1
  rxvldctr1_c_pipe/1 -> rxvldctr1/1(out_reg)
  rxeofctr1_del/1 -> rxeofctr1_r_pipe/1
  rxeofctr1_r_pipe/1 -> rxeofctr1_ctr/1
  rxeofctr1_ctr/1 -> rxeofctr1_c_pipe/1
  rxeofctr1_c_pipe/1 -> rxeofctr1/1(out_reg)
